simulink library "AEMS_Standard_Library"  (R2016b)
settings: Solver=ode45  StartTime=0.0  StopTime=10.0  RelTol=1e-3
undefined symbols (not defined in the file or in its folder): BkPY, carto, Cbx_extegr, Cbx_lpegrsys, Cbx_portegr, Cnx_bnk_nr_conf, Cnx_cyl_nr_conf, ConfigManagement, configuration_management, Cxx_dcm_io_tmr_end_xxxx, Cxx_dcm_rt_tmr_end, Cxx_DID_xxxx_IO_max, Cxx_DID_xxxx_IO_min, Cxx_egrhsofs, Cxx_vmaniegi, DEM_DEBOUNCE_FREEZE, DEM_DTR_CTL_INVISIBLE, DEM_DTR_CTL_NORMAL, Dem_DtrId2_XXX, Dem_DtrId3_XXX, Dem_DtrId4_XXX, Dem_DtrId5_XXX, Dem_DtrId6_XXX, Dem_DtrId7_XXX, Dem_DtrId8_XXX, Dem_DtrId9_XXX, Dem_DtrId_XXX, Dem_EnableConditionId2_XXX, Dem_EnableConditionId3_XXX, Dem_EnableConditionId4_XXX, Dem_EnableConditionId5_XXX, Dem_EnableConditionId6_XXX, Dem_EnableConditionId7_XXX, Dem_EnableConditionId8_XXX, Dem_EnableConditionId_XXX, Dem_EventId, Dem_EventId2_XXX, Dem_EventId3_XXX, Dem_EventId4_XXX, Dem_EventId5_XXX, Dem_EventId6_XXX, Dem_EventId7_XXX, Dem_EventId8_XXX, Dem_EventId9_XXX, Dem_EventId_Device_Faulttype, Dem_EventId_XXX, DEM_IUMPR_GENERAL_DENOMINATOR, DEM_OPCYC_IGNITION, Dem_RatioId2_XXX, Dem_RatioId3_XXX, Dem_RatioId4_XXX, Dem_RatioId5_XXX, Dem_RatioId6_XXX, Dem_RatioId7_XXX, Dem_RatioId8_XXX, Dem_RatioId_XXX, Dem_StorageConditionId2_XXX, Dem_StorageConditionId3_XXX, Dem_StorageConditionId4_XXX, Dem_StorageConditionId5_XXX ... (+65)
libraries: AEMS_Standard_Library x477, simulink x2
(part 12 of 39)

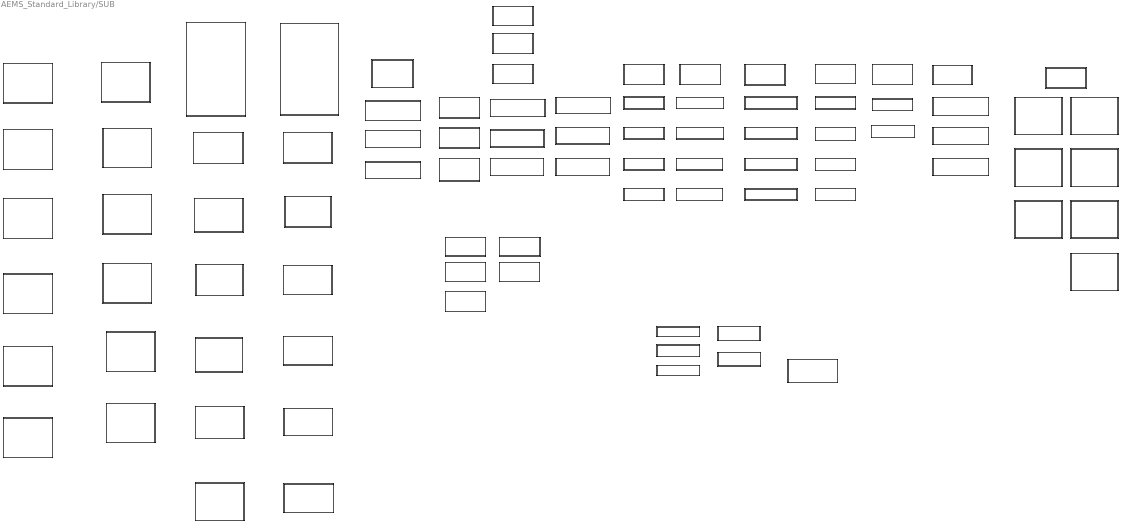
== system AEMS_Standard_Library/SUB ==
  AEMS_CONVERT_BUFFER_TO_FLP : Subsystem  Tag=[LIB]  mask(AEMS_CONVERT_BUFFER_TO_FLP){Resol=1, offset=0, DID_Datatype=int16}
      mask prompts: Resol "Resolution"; DID_Datatype "DID Datatype"
      mask help: This block converts the input buffer value to a float value.
      settings: AttributesFormatString=%<MaskType>\nResolution = %<Resol>\nOffset = %<offset>\nDIDType = %<DID_DataType>
      mask Help:
      | eval('path_lib=fileparts(which(''AEMS_Standard_Library''));');
      | doc_path = [path_lib'\help\AEMS_CONVERT_BUFFER_TO_FLP.pdf'];
      | eval('open(doc_path)');
      mask TypeOptions DID_Datatype: int8 | uint8 | int16 | uint16 | int32 | uint32
      mask Display:
      | try
      |     set_param(gcb,'MaskIconOpaque','opaque-with-ports');
      | catch
      |     set_param(gcb,'MaskIconOpaque','off');
      | end
      | 
      | disp('CONVERT_BUFFER_TO_FLP');
  AEMS_CONVERT_BYTE_TO_FLP : Subsystem  Tag=[LIB]  mask(AEMS_CONVERT_BYTE_TO_FLP){Resol=1, offset=0, DID_Datatype=int8}
      mask prompts: Resol "Resolution"; DID_Datatype "DID Datatype"
      mask help: This block is used to convert 1 byte data to corresponding floating point value based on resolution , offset & DID datatype.
      settings: AttributesFormatString=%<MaskType>\nResolution = %<Resol>\nOffset = %<offset>\nDIDType = %<DID_DataType>
      mask Help:
      | eval('path_lib=fileparts(which(''AEMS_Standard_Library''));');
      | doc_path = [path_lib'\help\AEMS_CONVERT_BYTE_TO_FLP'];
      | eval('open(doc_path)');
      mask TypeOptions DID_Datatype: int8 | uint8
      mask Display:
      | try
      |     set_param(gcb,'MaskIconOpaque','opaque-with-ports');
      | catch
      |     set_param(gcb,'MaskIconOpaque','off');
      | end
      | 
      | disp('CONVERT_BYTE_TO_FLP');
  AEMS_DEM_COUNTERBASEDDEBOUNCE : Subsystem  Tag=[LIB]  mask(AEMS_DEM_COUNTERBASEDDEBOUNCE){eventid=Dem_EventId_Device_Faulttype}
      mask prompts: eventid "Identifier of a diagnostic event (EventID)"
      mask help:
      | It  transmit the status Failed or Passed to the DEM. Accordingly, some bits of the UDS DTC status byte changes synchronously or asynchronously according to the configuration. Debounce is based on counter.
      |
      | -INPUTS-
      | conditionfulfilled: specifies whether the storage condition assigned to the StorageConditionID is fulfilled
      | prefailed: Monitor reports nonqualified test result pre-failed
      | prepassed: Monitor reports nonqualified test result pre-passed
      | reseteventdebounce: Freeze or reset the internal debounce counter/timer.
      | Dem Debounce Behavior: The event debounce counter will be frozen or reset (0 for FREEZE and 1 for RESET)
      | Dem Debounce Counter Failed Threshold: Defines the value of the internal debounce counter, which indicates the failed status.
      | Dem Debounce Counter Increment Step Size: Defines the incrementation  step size for counter (PREFAILED)
      | Dem Debounce Counter Jump Up: Activation of Jump-Up. True: activated. False: deactivated
      | Dem Debounce Counter Jump Up Value: Initialization value for the counter when PREFAILED
      | Dem Debounce Counter Passed Threshold: Defines the value of the internal debounce counter, which indicates the passed status.
      | Dem Debounce Counter Decrement Step Size: Defines the decrementation step for of counter (PREPASSED).
      | Dem Debounce Counter Jump Down: Activation of Jump-Down. True: Jump-Down activated
      | Dem Debounce Counter Jump Down Value: Initialization value for the counter when PREPASSED
      |
      | -OUTPUTS-
      | debouncevalue: Value of the debounce counter
      | failed: Diagnostic monitor reports an event Failed
      | passed: Diagnostic monitor reports an event passed
      |
      | -PARAMETERS-
      | EventID: Internal identifier of a diagnostic event. 0 is not a valid value.
      mask init:
      | eval([char(eventid) '= 0;'])
      | eventid_b = find_system(gcb,'LookUnderMasks','all','FollowLinks','on','Name','EventId_block');
      | set_param([eventid_b{:}],'Value',char(eventid));
      settings: AttributesFormatString=|
      | %<MaskType>
      | EventId: %<eventid>
  AEMS_DEM_COUNTER_BASED_DEBOUNCE_1D : Subsystem  Tag=[LIB]  Description=This subsystem is interface for self diagnosis standard calculated from similar condition and NG judgment.  mask(AEMS_DEM_COUNTER_BASED_DEBOUNCE_1D){eventid=Dem_EventId_Device_Faulttype, DemDebounceBehavior1=DEM_DEBOUNCE_FREEZE (0), DemCounterFailedThreshold=Cnx_dem_fail_thd_Device_Faulttype, DemCounterIncrementStepSize=Cnx_dem_pfail_inc_step_Device_Faulttype, DemCounterJumpUp=Cbx_dem_jmp_up_act_Device_Faulttype, DemCounterJumpUpValue=Cnx_dem_jmp_up_pfail_Device_Faulttype, DemCounterPassedThreshold=Cnx_dem_pass_thd_Device_Faulttype, DemCounterDecrementStepSize=Cnx_dem_ppass_dec_step_Device_Faulttype, DemCounterJumpDown=Cbx_dem_jmp_dwn_act_Device_Faulttype, DemCounterJumpDownValue=Cnx_dem_jmp_dwn_ppass_Device_Faulttype, DemCounterBypassFailure=Cbx_dem_byp_fail_Device_Faulttype}
      mask prompts: eventid "Identifier of a diagnostic event (EventId)"; DemDebounceBehavior1 "Dem Debounce Behavior"; DemCounterFailedThreshold "Dem Debounce Counter Failed Threshold"; DemCounterIncrementStepSize "Dem Debounce Counter Increment Step Size"; DemCounterJumpUp "Dem Debounce Counter Jump Up"; DemCounterJumpUpValue "Dem Debounce Counter Jump Up Value"; DemCounterPassedThreshold "Dem Debounce Counter Passed Threshold"; DemCounterDecrementStepSize "Dem Debounce Counter Decrement Step Size"; DemCounterJumpDown "Dem Debounce Counter Jump Down"; DemCounterJumpDownValue "Dem Debounce Counter Jump Down Value"; DemCounterBypassFailure "Dem Debounce Counter Bypass Failure"
      mask help:
      | It  transmit the status Failed or Passed to the DEM. Accordingly, some bits of the UDS DTC status byte changes synchronously or asynchronously according to the configuration. Debounce is based on counter.
      |
      | -INPUTS-
      | conditionfulfilled: specifies whether the storage condition assigned to the StorageConditionID is fulfilled
      | prefailed: Monitor reports nonqualified test result pre-failed
      | prepassed: Monitor reports nonqualified test result pre-passed
      | reseteventdebounce: Freeze or reset the internal debounce counter/timer.
      |
      | -OUTPUTS-
      | debouncevalue: Value of the debounce counter
      | failed: Diagnostic monitor reports an event Failed
      | passed: Diagnostic monitor reports an event passed
      |
      | -PARAMETERS-
      | Device: Device type
      | FaultType: Fault Type
      | EventID: Internal identifier of a diagnostic event. 0 is not a valid value.
      | Dem Debounce Behavior: The event debounce counter will be frozen or reset (0 for FREEZE and 1 for RESET)
      | Dem Debounce Counter Failed Threshold: Defines the value of the internal debounce counter, which indicates the failed status.
      | Dem Debounce Counter Increment Step Size: Defines the incrementation  step size for counter (PREFAILED)
      | Dem Debounce Counter Jump Up: Activation of Jump-Up. True: activated. False: deactivated
      | Dem Debounce Counter Jump Up Value: Initialization value for the counter when PREFAILED
      | Dem Debounce Counter Passed Threshold: Defines the value of the internal debounce counter, which indicates the passed status.
      | Dem Debounce Counter Decrement Step Size: Defines the decrementation step for of counter (PREPASSED).
      | Dem Debounce Counter Jump Down: Activation of Jump-Down. True: Jump-Down activated
      | Dem Debounce Counter Jump Down Value: Initialization value for the counter when PREPASSED
      mask init:
      | ThisBlk =gcb;
      | behaviorblk = [ThisBlk,'/DemDebounceBehavior'];
      | Bpath = [ThisBlk,'/AEMS_DEM_COUNTER_BASED_DEBOUNCE_CALL/AEMS_DEM_COUNTERBASEDDEBOUNCE'];
      | set_param(Bpath,'eventid',eventid);
      | if strcmpi(DemDebounceBehavior1,'DEM_DEBOUNCE_FREEZE (0)')
      |    set_param(behaviorblk,'Value','0');
      | elseif strcmpi(DemDebounceBehavior1,'DEM_DEBOUNCE_RESET (1)')
      |     set_param(behaviorblk,'Value','1');
      | end
      settings: AttributesFormatString=|
      | %<MaskType>
      | EventId: %<eventid>\nDem Debounce Behavior = %<DemDebounceBehavior1>\nDem Debounce Counter Failed Threshold = %<DemCounterFailedThreshold>\nDem Debounce Counter Increment Step Size = %<DemCounterIncrementStepSize>\nDem Debounce Counter Jump Up = %<DemCounterJumpUp>\nDem Debounce Counter Jump Up Value = %<DemCounterJumpUpValue>\nDem Debounce Counter Passed Threshold = %<DemCounterPassedThreshold>\nDem Debounce Counter Decrement Step Size = %<DemCounterDecrementStepSize>\nDem Debounce Counter Jump Down = %<DemCounterJumpDown>\nDem Debounce Counter Jump Down Value = %<DemCounterJumpDownValue>\nDem Debounce Counter Bypass Failure = %<DemCounterBypassFailure>
      mask Help:
      | eval('path_lib=fileparts(which(''AEMS_Standard_Library''));');
      | doc_path = [path_lib '\help\AEMS_DEM_COUNTER_BASED_DEBOUNCE.pdf'];
      | eval('open(doc_path)')
      mask TypeOptions DemDebounceBehavior1: DEM_DEBOUNCE_FREEZE (0) | DEM_DEBOUNCE_RESET (1)
  AEMS_DEM_COUNTER_BASED_DEBOUNCE_2D : Subsystem  Tag=[LIB]  Description=This subsystem is interface for self diagnosis standard calculated from similar condition and NG judgment.  mask(AEMS_DEM_COUNTER_BASED_DEBOUNCE_2D){eventid=Dem_EventId_Device_Faulttype, DemDebounceBehavior1=DEM_DEBOUNCE_FREEZE (0), DemDebounceBehavior2=DEM_DEBOUNCE_FREEZE (0), DemCounterFailedThreshold=Cnx_dem_fail_thd_Device_Faulttype, DemCounterIncrementStepSize=Cnx_dem_pfail_inc_step_Device_Faulttype, DemCounterJumpUp=Cbx_dem_jmp_up_act_Device_Faulttype, DemCounterJumpUpValue=Cnx_dem_jmp_up_pfail_Device_Faulttype, DemCounterPassedThreshold=Cnx_dem_pass_thd_Device_Faulttype, DemCounterDecrementStepSize=Cnx_dem_ppass_dec_step_Device_Faulttype, DemCounterJumpDown=Cbx_dem_jmp_dwn_act_Device_Faulttype, DemCounterJumpDownValue=Cnx_dem_jmp_dwn_ppass_Device_Faulttype, DemCounterBypassFailure=Cbx_dem_byp_fail_Device_Faulttype}
      mask prompts: eventid "Identifier of a diagnostic event (EventId)"; DemDebounceBehavior1 "Dem Debounce Behavior 1"; DemDebounceBehavior2 "Dem Debounce Behavior 2"; DemCounterFailedThreshold "Dem Debounce Counter Failed Threshold"; DemCounterIncrementStepSize "Dem Debounce Counter Increment Step Size"; DemCounterJumpUp "Dem Debounce Counter Jump Up"; DemCounterJumpUpValue "Dem Debounce Counter Jump Up Value"; DemCounterPassedThreshold "Dem Debounce Counter Passed Threshold"; DemCounterDecrementStepSize "Dem Debounce Counter Decrement Step Size"; DemCounterJumpDown "Dem Debounce Counter Jump Down"; DemCounterJumpDownValue "Dem Debounce Counter Jump Down Value"; DemCounterBypassFailure "Dem Debounce Counter Bypass Failure"
      mask help:
      | It  transmit the status Failed or Passed to the DEM. Accordingly, some bits of the UDS DTC status byte changes synchronously or asynchronously according to the configuration. Debounce is based on counter.
      |
      | -INPUTS-
      | conditionfulfilled: specifies whether the storage condition assigned to the StorageConditionID is fulfilled
      | prefailed: Monitor reports nonqualified test result pre-failed
      | prepassed: Monitor reports nonqualified test result pre-passed
      | reseteventdebounce: Freeze or reset the internal debounce counter/timer.
      |
      | -OUTPUTS-
      | debouncevalue: Value of the debounce counter
      | failed: Diagnostic monitor reports an event Failed
      | passed: Diagnostic monitor reports an event passed
      |
      | -PARAMETERS-
      | Device: Device type
      | FaultType: Fault Type
      | EventID: Internal identifier of a diagnostic event. 0 is not a valid value.
      | Dem Debounce Behavior: The event debounce counter will be frozen or reset (0 for FREEZE and 1 for RESET)
      | Dem Debounce Counter Failed Threshold: Defines the value of the internal debounce counter, which indicates the failed status.
      | Dem Debounce Counter Increment Step Size: Defines the incrementation  step size for counter (PREFAILED)
      | Dem Debounce Counter Jump Up: Activation of Jump-Up. True: activated. False: deactivated
      | Dem Debounce Counter Jump Up Value: Initialization value for the counter when PREFAILED
      | Dem Debounce Counter Passed Threshold: Defines the value of the internal debounce counter, which indicates the passed status.
      | Dem Debounce Counter Decrement Step Size: Defines the decrementation step for of counter (PREPASSED).
      | Dem Debounce Counter Jump Down: Activation of Jump-Down. True: Jump-Down activated
      | Dem Debounce Counter Jump Down Value: Initialization value for the counter when PREPASSED
      mask init:
      | ThisBlk =gcb;
      | DemDebounceBehaviors = {DemDebounceBehavior1,DemDebounceBehavior2};   
      | behaviorblk = [ThisBlk,'/DemDebounceBehavior'];
      | behaviorvector = '[';
      |     for cnt=1:2        
      |         cnt_str=num2str(cnt);
      |         Bpath = [ThisBlk,'/AEMS_DEM_COUNTER_BASED_DEBOUNCE_CALL',cnt_str,'/AEMS_DEM_COUNTERBASEDDEBOUNCE'];
      | %         set_param(Bpath,'eventid',[eventid,'_' cnt_str]);
      |         if (cnt==1)
      |             set_param(Bpath,'eventid',eventid);
      |         else
      |             Splitname=regexp(eventid,'_','all');
      |             New_EventId=insertBefore(eventid,Splitname(end),num2str(cnt));
      |             set_param(Bpath,'eventid',New_EventId);
      |         end
      |         if strcmpi(DemDebounceBehaviors{cnt},'DEM_DEBOUNCE_FREEZE (0)')
      |            behaviorvector= [behaviorvector,'0,'];
      |         else    
      |            behaviorvector= [behaviorvector,'1,'];        
      |         end
      |     end
      |     behaviorvector = behaviorvector(1:end-1);%Why end-1? I want to skip ',' for the last field.
      |     behaviorvector = [behaviorvector,']'];
      |     set_param(behaviorblk,'Value',behaviorvector);
      settings: AttributesFormatString=|
      | %<MaskType>
      | EventId: %<eventid>\nDem Debounce Behavior 1= %<DemDebounceBehavior1>\nDem Debounce Behavior 2= %<DemDebounceBehavior2>\nDem Debounce Counter Failed Threshold = %<DemCounterFailedThreshold>\nDem Debounce Counter Increment Step Size = %<DemCounterIncrementStepSize>\nDem Debounce Counter Jump Up = %<DemCounterJumpUp>\nDem Debounce Counter Jump Up Value = %<DemCounterJumpUpValue>\nDem Debounce Counter Passed Threshold = %<DemCounterPassedThreshold>\nDem Debounce Counter Decrement Step Size = %<DemCounterDecrementStepSize>\nDem Debounce Counter Jump Down = %<DemCounterJumpDown>\nDem Debounce Counter Jump Down Value = %<DemCounterJumpDownValue>\nDem Debounce Counter Bypass Failure = %<DemCounterBypassFailure>
      mask Help:
      | eval('path_lib=fileparts(which(''AEMS_Standard_Library''));');
      | doc_path = [path_lib '\help\AEMS_DEM_COUNTER_BASED_DEBOUNCE.pdf'];
      | eval('open(doc_path)')
      mask TypeOptions DemDebounceBehavior1: DEM_DEBOUNCE_FREEZE (0) | DEM_DEBOUNCE_RESET (1)
      mask TypeOptions DemDebounceBehavior2: DEM_DEBOUNCE_FREEZE (0) | DEM_DEBOUNCE_RESET (1)
  AEMS_DEM_COUNTER_BASED_DEBOUNCE_3D : Subsystem  Tag=[LIB]  Description=This subsystem is interface for self diagnosis standard calculated from similar condition and NG judgment.  mask(AEMS_DEM_COUNTER_BASED_DEBOUNCE_3D){eventid=Dem_EventId_Device_Faulttype, DemDebounceBehavior1=DEM_DEBOUNCE_FREEZE (0), DemDebounceBehavior2=DEM_DEBOUNCE_FREEZE (0), DemDebounceBehavior3=DEM_DEBOUNCE_FREEZE (0), DemCounterFailedThreshold=Cnx_dem_fail_thd_Device_Faulttype, DemCounterIncrementStepSize=Cnx_dem_pfail_inc_step_Device_Faulttype, DemCounterJumpUp=Cbx_dem_jmp_up_act_Device_Faulttype, DemCounterJumpUpValue=Cnx_dem_jmp_up_pfail_Device_Faulttype, DemCounterPassedThreshold=Cnx_dem_pass_thd_Device_Faulttype, DemCounterDecrementStepSize=Cnx_dem_ppass_dec_step_Device_Faulttype, DemCounterJumpDown=Cbx_dem_jmp_dwn_act_Device_Faulttype, DemCounterJumpDownValue=Cnx_dem_jmp_dwn_ppass_Device_Faulttype, DemCounterBypassFailure=Cbx_dem_byp_fail_Device_Faulttype}
      mask prompts: eventid "Identifier of a diagnostic event (EventId)"; DemDebounceBehavior1 "Dem Debounce Behavior 1"; DemDebounceBehavior2 "Dem Debounce Behavior 2"; DemDebounceBehavior3 "Dem Debounce Behavior 3"; DemCounterFailedThreshold "Dem Debounce Counter Failed Threshold"; DemCounterIncrementStepSize "Dem Debounce Counter Increment Step Size"; DemCounterJumpUp "Dem Debounce Counter Jump Up"; DemCounterJumpUpValue "Dem Debounce Counter Jump Up Value"; DemCounterPassedThreshold "Dem Debounce Counter Passed Threshold"; DemCounterDecrementStepSize "Dem Debounce Counter Decrement Step Size"; DemCounterJumpDown "Dem Debounce Counter Jump Down"; DemCounterJumpDownValue "Dem Debounce Counter Jump Down Value"; DemCounterBypassFailure "Dem Debounce Counter Bypass Failure"
      mask help:
      | It  transmit the status Failed or Passed to the DEM. Accordingly, some bits of the UDS DTC status byte changes synchronously or asynchronously according to the configuration. Debounce is based on counter.
      |
      | -INPUTS-
      | conditionfulfilled: specifies whether the storage condition assigned to the StorageConditionID is fulfilled
      | prefailed: Monitor reports nonqualified test result pre-failed
      | prepassed: Monitor reports nonqualified test result pre-passed
      | reseteventdebounce: Freeze or reset the internal debounce counter/timer.
      |
      | -OUTPUTS-
      | debouncevalue: Value of the debounce counter
      | failed: Diagnostic monitor reports an event Failed
      | passed: Diagnostic monitor reports an event passed
      |
      | -PARAMETERS-
      | Device: Device type
      | FaultType: Fault Type
      | EventID: Internal identifier of a diagnostic event. 0 is not a valid value.
      | Dem Debounce Behavior: The event debounce counter will be frozen or reset (0 for FREEZE and 1 for RESET)
      | Dem Debounce Counter Failed Threshold: Defines the value of the internal debounce counter, which indicates the failed status.
      | Dem Debounce Counter Increment Step Size: Defines the incrementation  step size for counter (PREFAILED)
      | Dem Debounce Counter Jump Up: Activation of Jump-Up. True: activated. False: deactivated
      | Dem Debounce Counter Jump Up Value: Initialization value for the counter when PREFAILED
      | Dem Debounce Counter Passed Threshold: Defines the value of the internal debounce counter, which indicates the passed status.
      | Dem Debounce Counter Decrement Step Size: Defines the decrementation step for of counter (PREPASSED).
      | Dem Debounce Counter Jump Down: Activation of Jump-Down. True: Jump-Down activated
      | Dem Debounce Counter Jump Down Value: Initialization value for the counter when PREPASSED
      mask init:
      | ThisBlk =gcb;
      | DemDebounceBehaviors = {DemDebounceBehavior1,DemDebounceBehavior2,DemDebounceBehavior3};   
      | behaviorblk = [ThisBlk,'/DemDebounceBehavior'];
      | behaviorvector = '[';
      |     for cnt=1:3        
      |         cnt_str=num2str(cnt);
      |         Bpath = [ThisBlk,'/AEMS_DEM_COUNTER_BASED_DEBOUNCE_CALL',cnt_str,'/AEMS_DEM_COUNTERBASEDDEBOUNCE'];
      |  %         set_param(Bpath,'eventid',[eventid,'_' cnt_str]);
      |         if (cnt==1)
      |             set_param(Bpath,'eventid',eventid);
      |         else
      |             Splitname=regexp(eventid,'_','all');
      |             New_EventId=insertBefore(eventid,Splitname(end),num2str(cnt));
      |             set_param(Bpath,'eventid',New_EventId);
      |         end
      |         if strcmpi(DemDebounceBehaviors{cnt},'DEM_DEBOUNCE_FREEZE (0)')
      |            behaviorvector= [behaviorvector,'0,'];
      |         else    
      |            behaviorvector= [behaviorvector,'1,'];        
      |         end
      |     end
      |     behaviorvector = behaviorvector(1:end-1);%Why end-1? I want to skip ',' for the last field.
      |     behaviorvector = [behaviorvector,']'];
      |     set_param(behaviorblk,'Value',behaviorvector);
      settings: AttributesFormatString=|
      | %<MaskType>
      | EventId: %<eventid>\nDem Debounce Behavior 1= %<DemDebounceBehavior1>\nDem Debounce Behavior 2= %<DemDebounceBehavior2>\nDem Debounce Behavior 3= %<DemDebounceBehavior3>\nDem Debounce Counter Failed Threshold = %<DemCounterFailedThreshold>\nDem Debounce Counter Increment Step Size = %<DemCounterIncrementStepSize>\nDem Debounce Counter Jump Up = %<DemCounterJumpUp>\nDem Debounce Counter Jump Up Value = %<DemCounterJumpUpValue>\nDem Debounce Counter Passed Threshold = %<DemCounterPassedThreshold>\nDem Debounce Counter Decrement Step Size = %<DemCounterDecrementStepSize>\nDem Debounce Counter Jump Down = %<DemCounterJumpDown>\nDem Debounce Counter Jump Down Value = %<DemCounterJumpDownValue>\nDem Debounce Counter Bypass Failure = %<DemCounterBypassFailure>
      mask Help:
      | eval('path_lib=fileparts(which(''AEMS_Standard_Library''));');
      | doc_path = [path_lib '\help\AEMS_DEM_COUNTER_BASED_DEBOUNCE.pdf'];
      | eval('open(doc_path)')
      mask TypeOptions DemDebounceBehavior1: DEM_DEBOUNCE_FREEZE (0) | DEM_DEBOUNCE_RESET (1)
      mask TypeOptions DemDebounceBehavior2: DEM_DEBOUNCE_FREEZE (0) | DEM_DEBOUNCE_RESET (1)
      mask TypeOptions DemDebounceBehavior3: DEM_DEBOUNCE_FREEZE (0) | DEM_DEBOUNCE_RESET (1)
  AEMS_DEM_COUNTER_BASED_DEBOUNCE_4D : Subsystem  Tag=[LIB]  Description=This subsystem is interface for self diagnosis standard calculated from similar condition and NG judgment.  mask(AEMS_DEM_COUNTER_BASED_DEBOUNCE_4D){eventid=Dem_EventId_Device_Faulttype, DemDebounceBehavior1=DEM_DEBOUNCE_FREEZE (0), DemDebounceBehavior2=DEM_DEBOUNCE_FREEZE (0), DemDebounceBehavior3=DEM_DEBOUNCE_FREEZE (0), DemDebounceBehavior4=DEM_DEBOUNCE_FREEZE (0), DemCounterFailedThreshold=Cnx_dem_fail_thd_Device_Faulttype, DemCounterIncrementStepSize=Cnx_dem_pfail_inc_step_Device_Faulttype, DemCounterJumpUp=Cbx_dem_jmp_up_act_Device_Faulttype, DemCounterJumpUpValue=Cnx_dem_jmp_up_pfail_Device_Faulttype, DemCounterPassedThreshold=Cnx_dem_pass_thd_Device_Faulttype, DemCounterDecrementStepSize=Cnx_dem_ppass_dec_step_Device_Faulttype, DemCounterJumpDown=Cbx_dem_jmp_dwn_act_Device_Faulttype, DemCounterJumpDownValue=Cnx_dem_jmp_dwn_ppass_Device_Faulttype, DemCounterBypassFailure=Cbx_dem_byp_fail_Device_Faulttype}
      mask prompts: eventid "Identifier of a diagnostic event (EventId)"; DemDebounceBehavior1 "Dem Debounce Behavior 1"; DemDebounceBehavior2 "Dem Debounce Behavior 2"; DemDebounceBehavior3 "Dem Debounce Behavior 3"; DemDebounceBehavior4 "Dem Debounce Behavior 4"; DemCounterFailedThreshold "Dem Debounce Counter Failed Threshold"; DemCounterIncrementStepSize "Dem Debounce Counter Increment Step Size"; DemCounterJumpUp "Dem Debounce Counter Jump Up"; DemCounterJumpUpValue "Dem Debounce Counter Jump Up Value"; DemCounterPassedThreshold "Dem Debounce Counter Passed Threshold"; DemCounterDecrementStepSize "Dem Debounce Counter Decrement Step Size"; DemCounterJumpDown "Dem Debounce Counter Jump Down"; DemCounterJumpDownValue "Dem Debounce Counter Jump Down Value"; DemCounterBypassFailure "Dem Debounce Counter Bypass Failure"
      mask help:
      | It  transmit the status Failed or Passed to the DEM. Accordingly, some bits of the UDS DTC status byte changes synchronously or asynchronously according to the configuration. Debounce is based on counter.
      |
      | -INPUTS-
      | conditionfulfilled: specifies whether the storage condition assigned to the StorageConditionID is fulfilled
      | prefailed: Monitor reports nonqualified test result pre-failed
      | prepassed: Monitor reports nonqualified test result pre-passed
      | reseteventdebounce: Freeze or reset the internal debounce counter/timer.
      |
      | -OUTPUTS-
      | debouncevalue: Value of the debounce counter
      | failed: Diagnostic monitor reports an event Failed
      | passed: Diagnostic monitor reports an event passed
      |
      | -PARAMETERS-
      | Device: Device type
      | FaultType: Fault Type
      | EventID: Internal identifier of a diagnostic event. 0 is not a valid value.
      | Dem Debounce Behavior: The event debounce counter will be frozen or reset (0 for FREEZE and 1 for RESET)
      | Dem Debounce Counter Failed Threshold: Defines the value of the internal debounce counter, which indicates the failed status.
      | Dem Debounce Counter Increment Step Size: Defines the incrementation  step size for counter (PREFAILED)
      | Dem Debounce Counter Jump Up: Activation of Jump-Up. True: activated. False: deactivated
      | Dem Debounce Counter Jump Up Value: Initialization value for the counter when PREFAILED
      | Dem Debounce Counter Passed Threshold: Defines the value of the internal debounce counter, which indicates the passed status.
      | Dem Debounce Counter Decrement Step Size: Defines the decrementation step for of counter (PREPASSED).
      | Dem Debounce Counter Jump Down: Activation of Jump-Down. True: Jump-Down activated
      | Dem Debounce Counter Jump Down Value: Initialization value for the counter when PREPASSED
      mask init:
      | ThisBlk =gcb;
      | DemDebounceBehaviors = {DemDebounceBehavior1,DemDebounceBehavior2,DemDebounceBehavior3,DemDebounceBehavior4};   
      | behaviorblk = [ThisBlk,'/DemDebounceBehavior'];
      | behaviorvector = '[';
      |     for cnt=1:4        
      |         cnt_str=num2str(cnt);
      |         Bpath = [ThisBlk,'/AEMS_DEM_COUNTER_BASED_DEBOUNCE_CALL',cnt_str,'/AEMS_DEM_COUNTERBASEDDEBOUNCE'];
      | %         set_param(Bpath,'eventid',[eventid,'_' cnt_str]);
      |         if (cnt==1)
      |             set_param(Bpath,'eventid',eventid);
      |         else
      |             Splitname=regexp(eventid,'_','all');
      |             New_EventId=insertBefore(eventid,Splitname(end),num2str(cnt));
      |             set_param(Bpath,'eventid',New_EventId);
      |         end
      |         if strcmpi(DemDebounceBehaviors{cnt},'DEM_DEBOUNCE_FREEZE (0)')
      |            behaviorvector= [behaviorvector,'0,'];
      |         else    
      |            behaviorvector= [behaviorvector,'1,'];        
      |         end
      |     end
      |     behaviorvector = behaviorvector(1:end-1);%Why end-1? I want to skip ',' for the last field.
      |     behaviorvector = [behaviorvector,']'];
      |     set_param(behaviorblk,'Value',behaviorvector);
      settings: AttributesFormatString=|
      | %<MaskType>
      | EventId: %<eventid>\nDem Debounce Behavior 1= %<DemDebounceBehavior1>\nDem Debounce Behavior 2= %<DemDebounceBehavior2>\nDem Debounce Behavior 3= %<DemDebounceBehavior3>\nDem Debounce Behavior 4= %<DemDebounceBehavior4>\nDem Debounce Counter Failed Threshold = %<DemCounterFailedThreshold>\nDem Debounce Counter Increment Step Size = %<DemCounterIncrementStepSize>\nDem Debounce Counter Jump Up = %<DemCounterJumpUp>\nDem Debounce Counter Jump Up Value = %<DemCounterJumpUpValue>\nDem Debounce Counter Passed Threshold = %<DemCounterPassedThreshold>\nDem Debounce Counter Decrement Step Size = %<DemCounterDecrementStepSize>\nDem Debounce Counter Jump Down = %<DemCounterJumpDown>\nDem Debounce Counter Jump Down Value = %<DemCounterJumpDownValue>\nDem Debounce Counter Bypass Failure = %<DemCounterBypassFailure>
      mask Help:
      | eval('path_lib=fileparts(which(''AEMS_Standard_Library''));');
      | doc_path = [path_lib '\help\AEMS_DEM_COUNTER_BASED_DEBOUNCE.pdf'];
      | eval('open(doc_path)')
      mask TypeOptions DemDebounceBehavior1: DEM_DEBOUNCE_FREEZE (0) | DEM_DEBOUNCE_RESET (1)
      mask TypeOptions DemDebounceBehavior2: DEM_DEBOUNCE_FREEZE (0) | DEM_DEBOUNCE_RESET (1)
      mask TypeOptions DemDebounceBehavior3: DEM_DEBOUNCE_FREEZE (0) | DEM_DEBOUNCE_RESET (1)
      mask TypeOptions DemDebounceBehavior4: DEM_DEBOUNCE_FREEZE (0) | DEM_DEBOUNCE_RESET (1)
  AEMS_DEM_COUNTER_BASED_DEBOUNCE_6D : Subsystem  Tag=[LIB]  Description=This subsystem is interface for self diagnosis standard calculated from similar condition and NG judgment.  mask(AEMS_DEM_COUNTER_BASED_DEBOUNCE_6D){eventid=Dem_EventId_Device_Faulttype, DemDebounceBehavior1=DEM_DEBOUNCE_FREEZE (0), DemDebounceBehavior2=DEM_DEBOUNCE_FREEZE (0), DemDebounceBehavior3=DEM_DEBOUNCE_FREEZE (0), DemDebounceBehavior4=DEM_DEBOUNCE_FREEZE (0), DemDebounceBehavior5=DEM_DEBOUNCE_FREEZE (0), DemDebounceBehavior6=DEM_DEBOUNCE_FREEZE (0), DemCounterFailedThreshold=Cnx_dem_fail_thd_Device_Faulttype, DemCounterIncrementStepSize=Cnx_dem_pfail_inc_step_Device_Faulttype, DemCounterJumpUp=Cbx_dem_jmp_up_act_Device_Faulttype, DemCounterJumpUpValue=Cnx_dem_jmp_up_pfail_Device_Faulttype, DemCounterPassedThreshold=Cnx_dem_pass_thd_Device_Faulttype, DemCounterDecrementStepSize=Cnx_dem_ppass_dec_step_Device_Faulttype, DemCounterJumpDown=Cbx_dem_jmp_dwn_act_Device_Faulttype, DemCounterJumpDownValue=Cnx_dem_jmp_dwn_ppass_Device_Faulttype, DemCounterBypassFailure=Cbx_dem_byp_fail_Device_Faulttype}
      mask prompts: eventid "Identifier of a diagnostic event (EventId)"; DemDebounceBehavior1 "Dem Debounce Behavior 1"; DemDebounceBehavior2 "Dem Debounce Behavior 2"; DemDebounceBehavior3 "Dem Debounce Behavior 3"; DemDebounceBehavior4 "Dem Debounce Behavior 4"; DemDebounceBehavior5 "Dem Debounce Behavior 5"; DemDebounceBehavior6 "Dem Debounce Behavior 6"; DemCounterFailedThreshold "Dem Debounce Counter Failed Threshold"; DemCounterIncrementStepSize "Dem Debounce Counter Increment Step Size"; DemCounterJumpUp "Dem Debounce Counter Jump Up"; DemCounterJumpUpValue "Dem Debounce Counter Jump Up Value"; DemCounterPassedThreshold "Dem Debounce Counter Passed Threshold"; DemCounterDecrementStepSize "Dem Debounce Counter Decrement Step Size"; DemCounterJumpDown "Dem Debounce Counter Jump Down"; DemCounterJumpDownValue "Dem Debounce Counter Jump Down Value"; DemCounterBypassFailure "Dem Debounce Counter Bypass Failure"
      mask help:
      | It  transmit the status Failed or Passed to the DEM. Accordingly, some bits of the UDS DTC status byte changes synchronously or asynchronously according to the configuration. Debounce is based on counter.
      |
      | -INPUTS-
      | conditionfulfilled: specifies whether the storage condition assigned to the StorageConditionID is fulfilled
      | prefailed: Monitor reports nonqualified test result pre-failed
      | prepassed: Monitor reports nonqualified test result pre-passed
      | reseteventdebounce: Freeze or reset the internal debounce counter/timer.
      |
      | -OUTPUTS-
      | debouncevalue: Value of the debounce counter
      | failed: Diagnostic monitor reports an event Failed
      | passed: Diagnostic monitor reports an event passed
      |
      | -PARAMETERS-
      | Device: Device type
      | FaultType: Fault Type
      | EventID: Internal identifier of a diagnostic event. 0 is not a valid value.
      | Dem Debounce Behavior: The event debounce counter will be frozen or reset (0 for FREEZE and 1 for RESET)
      | Dem Debounce Counter Failed Threshold: Defines the value of the internal debounce counter, which indicates the failed status.
      | Dem Debounce Counter Increment Step Size: Defines the incrementation  step size for counter (PREFAILED)
      | Dem Debounce Counter Jump Up: Activation of Jump-Up. True: activated. False: deactivated
      | Dem Debounce Counter Jump Up Value: Initialization value for the counter when PREFAILED
      | Dem Debounce Counter Passed Threshold: Defines the value of the internal debounce counter, which indicates the passed status.
      | Dem Debounce Counter Decrement Step Size: Defines the decrementation step for of counter (PREPASSED).
      | Dem Debounce Counter Jump Down: Activation of Jump-Down. True: Jump-Down activated
      | Dem Debounce Counter Jump Down Value: Initialization value for the counter when PREPASSED
      mask init:
      | ThisBlk =gcb;
      | DemDebounceBehaviors = {DemDebounceBehavior1,DemDebounceBehavior2,DemDebounceBehavior3,DemDebounceBehavior4,DemDebounceBehavior5,DemDebounceBehavior6};   
      | behaviorblk = [ThisBlk,'/DemDebounceBehavior'];
      | behaviorvector = '[';
      |     for cnt=1:6        
      |         cnt_str=num2str(cnt);
      |         Bpath = [ThisBlk,'/AEMS_DEM_COUNTER_BASED_DEBOUNCE_CALL',cnt_str,'/AEMS_DEM_COUNTERBASEDDEBOUNCE'];
      | %         set_param(Bpath,'eventid',[eventid,'_' cnt_str]);
      |         if (cnt==1)
      |             set_param(Bpath,'eventid',eventid);
      |         else
      |             Splitname=regexp(eventid,'_','all');
      |             New_EventId=insertBefore(eventid,Splitname(end),num2str(cnt));
      |             set_param(Bpath,'eventid',New_EventId);
      |         end
      |         if strcmpi(DemDebounceBehaviors{cnt},'DEM_DEBOUNCE_FREEZE (0)')
      |            behaviorvector= [behaviorvector,'0,'];
      |         else    
      |            behaviorvector= [behaviorvector,'1,'];        
      |         end
      |     end
      |     behaviorvector = behaviorvector(1:end-1);%Why end-1? I want to skip ',' for the last field.
      |     behaviorvector = [behaviorvector,']'];
      |     set_param(behaviorblk,'Value',behaviorvector);
      settings: AttributesFormatString=|
      | %<MaskType>
      | EventId: %<eventid>\nDem Debounce Behavior 1= %<DemDebounceBehavior1>\nDem Debounce Behavior 2= %<DemDebounceBehavior2>\nDem Debounce Behavior 3= %<DemDebounceBehavior3>\nDem Debounce Behavior 4= %<DemDebounceBehavior4>\nDem Debounce Behavior 5= %<DemDebounceBehavior5>\nDem Debounce Behavior 6= %<DemDebounceBehavior6>\nDem Debounce Counter Failed Threshold = %<DemCounterFailedThreshold>\nDem Debounce Counter Increment Step Size = %<DemCounterIncrementStepSize>\nDem Debounce Counter Jump Up = %<DemCounterJumpUp>\nDem Debounce Counter Jump Up Value = %<DemCounterJumpUpValue>\nDem Debounce Counter Passed Threshold = %<DemCounterPassedThreshold>\nDem Debounce Counter Decrement Step Size = %<DemCounterDecrementStepSize>\nDem Debounce Counter Jump Down = %<DemCounterJumpDown>\nDem Debounce Counter Jump Down Value = %<DemCounterJumpDownValue>\nDem Debounce Counter Bypass Failure = %<DemCounterBypassFailure>
      mask Help:
      | eval('path_lib=fileparts(which(''AEMS_Standard_Library''));');
      | doc_path = [path_lib '\help\AEMS_DEM_COUNTER_BASED_DEBOUNCE.pdf'];
      | eval('open(doc_path)')
      mask TypeOptions DemDebounceBehavior1: DEM_DEBOUNCE_FREEZE (0) | DEM_DEBOUNCE_RESET (1)
      mask TypeOptions DemDebounceBehavior2: DEM_DEBOUNCE_FREEZE (0) | DEM_DEBOUNCE_RESET (1)
      mask TypeOptions DemDebounceBehavior3: DEM_DEBOUNCE_FREEZE (0) | DEM_DEBOUNCE_RESET (1)
      mask TypeOptions DemDebounceBehavior4: DEM_DEBOUNCE_FREEZE (0) | DEM_DEBOUNCE_RESET (1)
      mask TypeOptions DemDebounceBehavior5: DEM_DEBOUNCE_FREEZE (0) | DEM_DEBOUNCE_RESET (1)
      mask TypeOptions DemDebounceBehavior6: DEM_DEBOUNCE_FREEZE (0) | DEM_DEBOUNCE_RESET (1)
  AEMS_DEM_COUNTER_BASED_DEBOUNCE_8D : Subsystem  Tag=[LIB]  Description=This subsystem is interface for self diagnosis standard calculated from similar condition and NG judgment.  mask(AEMS_DEM_COUNTER_BASED_DEBOUNCE_8D){eventid=Dem_EventId_Device_Faulttype, DemDebounceBehavior1=DEM_DEBOUNCE_FREEZE (0), DemDebounceBehavior2=DEM_DEBOUNCE_FREEZE (0), DemDebounceBehavior3=DEM_DEBOUNCE_FREEZE (0), DemDebounceBehavior4=DEM_DEBOUNCE_FREEZE (0), DemDebounceBehavior5=DEM_DEBOUNCE_FREEZE (0), DemDebounceBehavior6=DEM_DEBOUNCE_FREEZE (0), DemDebounceBehavior7=DEM_DEBOUNCE_FREEZE (0), DemDebounceBehavior8=DEM_DEBOUNCE_FREEZE (0), DemCounterFailedThreshold=Cnx_dem_fail_thd_Device_Faulttype, DemCounterIncrementStepSize=Cnx_dem_pfail_inc_step_Device_Faulttype, DemCounterJumpUp=Cbx_dem_jmp_up_act_Device_Faulttype, DemCounterJumpUpValue=Cnx_dem_jmp_up_pfail_Device_Faulttype, DemCounterPassedThreshold=Cnx_dem_pass_thd_Device_Faulttype, DemCounterDecrementStepSize=Cnx_dem_ppass_dec_step_Device_Faulttype, DemCounterJumpDown=Cbx_dem_jmp_dwn_act_Device_Faulttype, DemCounterJumpDownValue=Cnx_dem_jmp_dwn_ppass_Device_Faulttype, DemCounterBypassFailure=Cbx_dem_byp_fail_Device_Faulttype}
      mask prompts: eventid "Identifier of a diagnostic event (EventId)"; DemDebounceBehavior1 "Dem Debounce Behavior 1"; DemDebounceBehavior2 "Dem Debounce Behavior 2"; DemDebounceBehavior3 "Dem Debounce Behavior 3"; DemDebounceBehavior4 "Dem Debounce Behavior 4"; DemDebounceBehavior5 "Dem Debounce Behavior 5"; DemDebounceBehavior6 "Dem Debounce Behavior 6"; DemDebounceBehavior7 "Dem Debounce Behavior 7"; DemDebounceBehavior8 "Dem Debounce Behavior 8"; DemCounterFailedThreshold "Dem Debounce Counter Failed Threshold"; DemCounterIncrementStepSize "Dem Debounce Counter Increment Step Size"; DemCounterJumpUp "Dem Debounce Counter Jump Up"; DemCounterJumpUpValue "Dem Debounce Counter Jump Up Value"; DemCounterPassedThreshold "Dem Debounce Counter Passed Threshold"; DemCounterDecrementStepSize "Dem Debounce Counter Decrement Step Size"; DemCounterJumpDown "Dem Debounce Counter Jump Down"; DemCounterJumpDownValue "Dem Debounce Counter Jump Down Value"; DemCounterBypassFailure "Dem Debounce Counter Bypass Failure"
      mask help:
      | It  transmit the status Failed or Passed to the DEM. Accordingly, some bits of the UDS DTC status byte changes synchronously or asynchronously according to the configuration. Debounce is based on counter.
      |
      | -INPUTS-
      | conditionfulfilled: specifies whether the storage condition assigned to the StorageConditionID is fulfilled
      | prefailed: Monitor reports nonqualified test result pre-failed
      | prepassed: Monitor reports nonqualified test result pre-passed
      | reseteventdebounce: Freeze or reset the internal debounce counter/timer.
      |
      | -OUTPUTS-
      | debouncevalue: Value of the debounce counter
      | failed: Diagnostic monitor reports an event Failed
      | passed: Diagnostic monitor reports an event passed
      |
      | -PARAMETERS-
      | Device: Device type
      | FaultType: Fault Type
      | EventID: Internal identifier of a diagnostic event. 0 is not a valid value.
      | Dem Debounce Behavior: The event debounce counter will be frozen or reset (0 for FREEZE and 1 for RESET)
      | Dem Debounce Counter Failed Threshold: Defines the value of the internal debounce counter, which indicates the failed status.
      | Dem Debounce Counter Increment Step Size: Defines the incrementation  step size for counter (PREFAILED)
      | Dem Debounce Counter Jump Up: Activation of Jump-Up. True: activated. False: deactivated
      | Dem Debounce Counter Jump Up Value: Initialization value for the counter when PREFAILED
      | Dem Debounce Counter Passed Threshold: Defines the value of the internal debounce counter, which indicates the passed status.
      | Dem Debounce Counter Decrement Step Size: Defines the decrementation step for of counter (PREPASSED).
      | Dem Debounce Counter Jump Down: Activation of Jump-Down. True: Jump-Down activated
      | Dem Debounce Counter Jump Down Value: Initialization value for the counter when PREPASSED
      mask init:
      | ThisBlk =gcb;
      | DemDebounceBehaviors = {DemDebounceBehavior1,DemDebounceBehavior2,DemDebounceBehavior3,DemDebounceBehavior4,DemDebounceBehavior5,DemDebounceBehavior6,DemDebounceBehavior7,DemDebounceBehavior8};   
      | behaviorblk = [ThisBlk,'/DemDebounceBehavior'];
      | behaviorvector = '[';
      |     for cnt=1:8        
      |         cnt_str=num2str(cnt);
      |         Bpath = [ThisBlk,'/AEMS_DEM_COUNTER_BASED_DEBOUNCE_CALL',cnt_str,'/AEMS_DEM_COUNTERBASEDDEBOUNCE'];
      | %         set_param(Bpath,'eventid',[eventid,'_' cnt_str]);
      |         if (cnt==1)
      |             set_param(Bpath,'eventid',eventid);
      |         else
      |             Splitname=regexp(eventid,'_','all');
      |             New_EventId=insertBefore(eventid,Splitname(end),num2str(cnt));
      |             set_param(Bpath,'eventid',New_EventId);
      |         end
      |         if strcmpi(DemDebounceBehaviors{cnt},'DEM_DEBOUNCE_FREEZE (0)')
      |            behaviorvector= [behaviorvector,'0,'];
      |         else    
      |            behaviorvector= [behaviorvector,'1,'];        
      |         end
      |     end
      |     behaviorvector = behaviorvector(1:end-1);%Why end-1? I want to skip ',' for the last field.
      |     behaviorvector = [behaviorvector,']'];
      |     set_param(behaviorblk,'Value',behaviorvector);
      settings: AttributesFormatString=|
      | %<MaskType>
      | EventId: %<eventid>\nDem Debounce Behavior 1= %<DemDebounceBehavior1>\nDem Debounce Behavior 2= %<DemDebounceBehavior2>\nDem Debounce Behavior 3= %<DemDebounceBehavior3>\nDem Debounce Behavior 4= %<DemDebounceBehavior4>\nDem Debounce Behavior 5= %<DemDebounceBehavior5>\nDem Debounce Behavior 6= %<DemDebounceBehavior6>\nDem Debounce Behavior 7= %<DemDebounceBehavior7>\nDem Debounce Behavior 8= %<DemDebounceBehavior8>\nDem Debounce Counter Failed Threshold = %<DemCounterFailedThreshold>\nDem Debounce Counter Increment Step Size = %<DemCounterIncrementStepSize>\nDem Debounce Counter Jump Up = %<DemCounterJumpUp>\nDem Debounce Counter Jump Up Value = %<DemCounterJumpUpValue>\nDem Debounce Counter Passed Threshold = %<DemCounterPassedThreshold>\nDem Debounce Counter Decrement Step Size = %<DemCounterDecrementStepSize>\nDem Debounce Counter Jump Down = %<DemCounterJumpDown>\nDem Debounce Counter Jump Down Value = %<DemCounterJumpDownValue>\nDem Debounce Counter Bypass Failure = %<DemCounterBypassFailure>
      mask Help:
      | eval('path_lib=fileparts(which(''AEMS_Standard_Library''));');
      | doc_path = [path_lib '\help\AEMS_DEM_COUNTER_BASED_DEBOUNCE.pdf'];
      | eval('open(doc_path)')
      mask TypeOptions DemDebounceBehavior1: DEM_DEBOUNCE_FREEZE (0) | DEM_DEBOUNCE_RESET (1)
      mask TypeOptions DemDebounceBehavior2: DEM_DEBOUNCE_FREEZE (0) | DEM_DEBOUNCE_RESET (1)
      mask TypeOptions DemDebounceBehavior3: DEM_DEBOUNCE_FREEZE (0) | DEM_DEBOUNCE_RESET (1)
      mask TypeOptions DemDebounceBehavior4: DEM_DEBOUNCE_FREEZE (0) | DEM_DEBOUNCE_RESET (1)
      mask TypeOptions DemDebounceBehavior5: DEM_DEBOUNCE_FREEZE (0) | DEM_DEBOUNCE_RESET (1)
      mask TypeOptions DemDebounceBehavior6: DEM_DEBOUNCE_FREEZE (0) | DEM_DEBOUNCE_RESET (1)
      mask TypeOptions DemDebounceBehavior7: DEM_DEBOUNCE_FREEZE (0) | DEM_DEBOUNCE_RESET (1)
      mask TypeOptions DemDebounceBehavior8: DEM_DEBOUNCE_FREEZE (0) | DEM_DEBOUNCE_RESET (1)
  AEMS_DEM_COUNTER_BASED_DEBOUNCE_THRSHOLD_DYN_1D : Subsystem  Tag=[LIB]  Description=This subsystem is interface for self diagnosis standard calculated from similar condition and NG judgment.  mask(AEMS_DEM_COUNTER_BASED_DEBOUNCE_THRSHOLD_DYN_1D){eventid=Dem_EventId_Device_Faulttype, DemDebounceBehavior1=DEM_DEBOUNCE_FREEZE (0), DemCounterIncrementStepSize=Cnx_dem_pfail_inc_step_Device_Faulttype, DemCounterJumpUp=Cbx_dem_jmp_up_act_Device_Faulttype, DemCounterJumpUpValue=Cnx_dem_jmp_up_pfail_Device_Faulttype, DemCounterDecrementStepSize=Cnx_dem_ppass_dec_step_Device_Faulttype, DemCounterJumpDown=Cbx_dem_jmp_dwn_act_Device_Faulttype, DemCounterJumpDownValue=Cnx_dem_jmp_dwn_ppass_Device_Faulttype, DemCounterBypassFailure=Cbx_dem_byp_fail_Device_Faulttype}
      mask prompts: eventid "Identifier of a diagnostic event (EventId)"; DemDebounceBehavior1 "Dem Debounce Behavior"; DemCounterIncrementStepSize "Dem Debounce Counter Increment Step Size"; DemCounterJumpUp "Dem Debounce Counter Jump Up"; DemCounterJumpUpValue "Dem Debounce Counter Jump Up Value"; DemCounterDecrementStepSize "Dem Debounce Counter Decrement Step Size"; DemCounterJumpDown "Dem Debounce Counter Jump Down"; DemCounterJumpDownValue "Dem Debounce Counter Jump Down Value"; DemCounterBypassFailure "Dem Debounce Counter Bypass Failure"
      mask help:
      | It  transmit the status Failed or Passed to the DEM. Accordingly, some bits of the UDS DTC status byte changes synchronously or asynchronously according to the configuration. Debounce is based on counter.
      |
      | -INPUTS-
      | conditionfulfilled: specifies whether the storage condition assigned to the StorageConditionID is fulfilled
      | prefailed: Monitor reports nonqualified test result pre-failed
      | prepassed: Monitor reports nonqualified test result pre-passed
      | failedthreshold: Defines the value of the internal debounce counter, which indicates the failed status.
      | passedthreshold: Defines the value of the internal debounce counter, which indicates the passed status.
      | reseteventdebounce: Freeze or reset the internal debounce counter/timer.
      |
      | -OUTPUTS-
      | debouncevalue: Value of the debounce counter
      | failed: Diagnostic monitor reports an event Failed
      | passed: Diagnostic monitor reports an event passed
      |
      | -PARAMETERS-
      | EventID: Internal identifier of a diagnostic event. 0 is not a valid value.
      | Dem Debounce Behavior: The event debounce counter will be frozen or reset (0 for FREEZE and 1 for RESET)
      | Dem Debounce Counter Increment Step Size: Defines the incrementation  step size for counter (PREFAILED)
      | Dem Debounce Counter Jump Up: Activation of Jump-Up. True: activated. False: deactivated
      | Dem Debounce Counter Jump Up Value: Initialization value for the counter when PREFAILED
      | Dem Debounce Counter Decrement Step Size: Defines the decrementation step for of counter (PREPASSED).
      | Dem Debounce Counter Jump Down: Activation of Jump-Down. True: Jump-Down activated
      | Dem Debounce Counter Jump Down Value: Initialization value for the counter when PREPASSED
      mask init:
      | ThisBlk =gcb;
      | behaviorblk = [ThisBlk,'/DemDebounceBehavior'];
      | Bpath = [ThisBlk,'/AEMS_DEM_COUNTER_BASED_DEBOUNCE_THRSHOLD_DYN_CALL/AEMS_DEM_COUNTERBASEDDEBOUNCE'];
      | set_param(Bpath,'eventid',eventid);
      | if strcmpi(DemDebounceBehavior1,'DEM_DEBOUNCE_FREEZE (0)')
      |    set_param(behaviorblk,'Value','0');
      | elseif strcmpi(DemDebounceBehavior1,'DEM_DEBOUNCE_RESET (1)')
      |     set_param(behaviorblk,'Value','1');
      | end
      settings: AttributesFormatString=|
      | %<MaskType>\nEventId: %<eventid>
      | Dem Debounce Behavior = %<DemDebounceBehavior1>
      | Dem Debounce Counter Increment Step Size = %<DemCounterIncrementStepSize>
      | Dem Debounce Counter Jump Up = %<DemCounterJumpUp>
      | Dem Debounce Counter Jump Up Value = %<DemCounterJumpUpValue>
      | Dem Debounce Counter Decrement Step Size = %<DemCounterDecrementStepSize>
      | Dem Debounce Counter Jump Down = %<DemCounterJumpDown>
      | Dem Debounce Counter Jump Down Value = %<DemCounterJumpDownValue>
      | Dem Debounce Counter Bypass Failure = %<DemCounterBypassFailure>
      mask Help:
      | eval('path_lib=fileparts(which(''AEMS_Standard_Library''));');
      | doc_path = [path_lib '\help\AEMS_DEM_COUNTER_BASED_DEBOUNCE_THRSHOLD_DYN.pdf'];
      | eval('open(doc_path)')
      mask TypeOptions DemDebounceBehavior1: DEM_DEBOUNCE_FREEZE (0) | DEM_DEBOUNCE_RESET (1)
  AEMS_DEM_COUNTER_BASED_DEBOUNCE_THRSHOLD_DYN_2D : Subsystem  Tag=[LIB]  Description=This subsystem is interface for self diagnosis standard calculated from similar condition and NG judgment.  mask(AEMS_DEM_COUNTER_BASED_DEBOUNCE_THRSHOLD_DYN_2D){eventid=Dem_EventId_Device_Faulttype, DemDebounceBehavior1=DEM_DEBOUNCE_FREEZE (0), DemDebounceBehavior2=DEM_DEBOUNCE_FREEZE (0), DemCounterIncrementStepSize=Cnx_dem_pfail_inc_step_Device_Faulttype, DemCounterJumpUp=Cbx_dem_jmp_up_act_Device_Faulttype, DemCounterJumpUpValue=Cnx_dem_jmp_up_pfail_Device_Faulttype, DemCounterDecrementStepSize=Cnx_dem_ppass_dec_step_Device_Faulttype, DemCounterJumpDown=Cbx_dem_jmp_dwn_act_Device_Faulttype, DemCounterJumpDownValue=Cnx_dem_jmp_dwn_ppass_Device_Faulttype, DemCounterBypassFailure=Cbx_dem_byp_fail_Device_Faulttype}
      mask prompts: eventid "Identifier of a diagnostic event (EventId)"; DemDebounceBehavior1 "Dem Debounce Behavior 1"; DemDebounceBehavior2 "Dem Debounce Behavior 2"; DemCounterIncrementStepSize "Dem Debounce Counter Increment Step Size"; DemCounterJumpUp "Dem Debounce Counter Jump Up"; DemCounterJumpUpValue "Dem Debounce Counter Jump Up Value"; DemCounterDecrementStepSize "Dem Debounce Counter Decrement Step Size"; DemCounterJumpDown "Dem Debounce Counter Jump Down"; DemCounterJumpDownValue "Dem Debounce Counter Jump Down Value"; DemCounterBypassFailure "Dem Debounce Counter Bypass Failure"
      mask help:
      | It  transmit the status Failed or Passed to the DEM. Accordingly, some bits of the UDS DTC status byte changes synchronously or asynchronously according to the configuration. Debounce is based on counter.
      |
      | -INPUTS-
      | conditionfulfilled: specifies whether the storage condition assigned to the StorageConditionID is fulfilled
      | prefailed: Monitor reports nonqualified test result pre-failed
      | prepassed: Monitor reports nonqualified test result pre-passed
      | failedthreshold: Defines the value of the internal debounce counter, which indicates the failed status.
      | passedthreshold: Defines the value of the internal debounce counter, which indicates the passed status.
      | reseteventdebounce: Freeze or reset the internal debounce counter/timer.
      |
      | -OUTPUTS-
      | debouncevalue: Value of the debounce counter
      | failed: Diagnostic monitor reports an event Failed
      | passed: Diagnostic monitor reports an event passed
      |
      | -PARAMETERS-
      | EventID: Internal identifier of a diagnostic event. 0 is not a valid value.
      | Dem Debounce Behavior: The event debounce counter will be frozen or reset (0 for FREEZE and 1 for RESET)
      | Dem Debounce Counter Increment Step Size: Defines the incrementation  step size for counter (PREFAILED)
      | Dem Debounce Counter Jump Up: Activation of Jump-Up. True: activated. False: deactivated
      | Dem Debounce Counter Jump Up Value: Initialization value for the counter when PREFAILED
      | Dem Debounce Counter Decrement Step Size: Defines the decrementation step for of counter (PREPASSED).
      | Dem Debounce Counter Jump Down: Activation of Jump-Down. True: Jump-Down activated
      | Dem Debounce Counter Jump Down Value: Initialization value for the counter when PREPASSED
      mask init:
      | ThisBlk =gcb;
      | DemDebounceBehaviors = {DemDebounceBehavior1,DemDebounceBehavior2};
      | behaviorblk = [ThisBlk,'/DemDebounceBehavior'];
      | behaviorvector = '[';
      | for cnt=1:2
      |     cnt_str=num2str(cnt);
      |     Bpath = [ThisBlk,'/AEMS_DEM_COUNTER_BASED_DEBOUNCE_THRSHOLD_DYN_CALL',cnt_str,'/AEMS_DEM_COUNTERBASEDDEBOUNCE'];
      | %     set_param(Bpath,'eventid',[eventid,'_' cnt_str]);
      |     if (cnt==1)
      |         set_param(Bpath,'eventid',eventid);
      |     else
      |         Splitname=regexp(eventid,'_','all');
      |         New_EventId=insertBefore(eventid,Splitname(end),num2str(cnt));
      |         set_param(Bpath,'eventid',New_EventId);
      |     end
      |     if strcmpi(DemDebounceBehaviors{cnt},'DEM_DEBOUNCE_FREEZE (0)')
      |         behaviorvector= [behaviorvector,'0,'];
      |     else
      |         behaviorvector= [behaviorvector,'1,'];
      |     end
      | end
      | behaviorvector = behaviorvector(1:end-1);%Why end-1? I want to skip ',' for the last field.
      | behaviorvector = [behaviorvector,']'];
      | set_param(behaviorblk,'Value',behaviorvector);
      settings: AttributesFormatString=|
      | %<MaskType>\nEventId: %<eventid>
      | Dem Debounce Behavior 1 = %<DemDebounceBehavior1>
      | Dem Debounce Behavior 2 = %<DemDebounceBehavior2>
      | Dem Debounce Counter Increment Step Size = %<DemCounterIncrementStepSize>
      | Dem Debounce Counter Jump Up = %<DemCounterJumpUp>
      | Dem Debounce Counter Jump Up Value = %<DemCounterJumpUpValue>
      | Dem Debounce Counter Decrement Step Size = %<DemCounterDecrementStepSize>
      | Dem Debounce Counter Jump Down = %<DemCounterJumpDown>
      | Dem Debounce Counter Jump Down Value = %<DemCounterJumpDownValue>
      | Dem Debounce Counter Bypass Failure = %<DemCounterBypassFailure>
      mask Help:
      | eval('path_lib=fileparts(which(''AEMS_Standard_Library''));');
      | doc_path = [path_lib '\help\AEMS_DEM_COUNTER_BASED_DEBOUNCE_THRSHOLD_DYN.pdf'];
      | eval('open(doc_path)')
      mask TypeOptions DemDebounceBehavior1: DEM_DEBOUNCE_FREEZE (0) | DEM_DEBOUNCE_RESET (1)
      mask TypeOptions DemDebounceBehavior2: DEM_DEBOUNCE_FREEZE (0) | DEM_DEBOUNCE_RESET (1)
  AEMS_DEM_COUNTER_BASED_DEBOUNCE_THRSHOLD_DYN_3D : Subsystem  Tag=[LIB]  Description=This subsystem is interface for self diagnosis standard calculated from similar condition and NG judgment.  mask(AEMS_DEM_COUNTER_BASED_DEBOUNCE_THRSHOLD_DYN_3D){eventid=Dem_EventId_Device_Faulttype, DemDebounceBehavior1=DEM_DEBOUNCE_FREEZE (0), DemDebounceBehavior2=DEM_DEBOUNCE_FREEZE (0), DemDebounceBehavior3=DEM_DEBOUNCE_FREEZE (0), DemCounterIncrementStepSize=Cnx_dem_pfail_inc_step_Device_Faulttype, DemCounterJumpUp=Cbx_dem_jmp_up_act_Device_Faulttype, DemCounterJumpUpValue=Cnx_dem_jmp_up_pfail_Device_Faulttype, DemCounterDecrementStepSize=Cnx_dem_ppass_dec_step_Device_Faulttype, DemCounterJumpDown=Cbx_dem_jmp_dwn_act_Device_Faulttype, DemCounterJumpDownValue=Cnx_dem_jmp_dwn_ppass_Device_Faulttype, DemCounterBypassFailure=Cbx_dem_byp_fail_Device_Faulttype}
      mask prompts: eventid "Identifier of a diagnostic event (EventId)"; DemDebounceBehavior1 "Dem Debounce Behavior 1"; DemDebounceBehavior2 "Dem Debounce Behavior 2"; DemDebounceBehavior3 "Dem Debounce Behavior 3"; DemCounterIncrementStepSize "Dem Debounce Counter Increment Step Size"; DemCounterJumpUp "Dem Debounce Counter Jump Up"; DemCounterJumpUpValue "Dem Debounce Counter Jump Up Value"; DemCounterDecrementStepSize "Dem Debounce Counter Decrement Step Size"; DemCounterJumpDown "Dem Debounce Counter Jump Down"; DemCounterJumpDownValue "Dem Debounce Counter Jump Down Value"; DemCounterBypassFailure "Dem Debounce Counter Bypass Failure"
      mask help:
      | It  transmit the status Failed or Passed to the DEM. Accordingly, some bits of the UDS DTC status byte changes synchronously or asynchronously according to the configuration. Debounce is based on counter.
      |
      | -INPUTS-
      | conditionfulfilled: specifies whether the storage condition assigned to the StorageConditionID is fulfilled
      | prefailed: Monitor reports nonqualified test result pre-failed
      | prepassed: Monitor reports nonqualified test result pre-passed
      | failedthreshold: Defines the value of the internal debounce counter, which indicates the failed status.
      | passedthreshold: Defines the value of the internal debounce counter, which indicates the passed status.
      | reseteventdebounce: Freeze or reset the internal debounce counter/timer.
      |
      | -OUTPUTS-
      | debouncevalue: Value of the debounce counter
      | failed: Diagnostic monitor reports an event Failed
      | passed: Diagnostic monitor reports an event passed
      |
      | -PARAMETERS-
      | EventID: Internal identifier of a diagnostic event. 0 is not a valid value.
      | Dem Debounce Behavior: The event debounce counter will be frozen or reset (0 for FREEZE and 1 for RESET)
      | Dem Debounce Counter Increment Step Size: Defines the incrementation  step size for counter (PREFAILED)
      | Dem Debounce Counter Jump Up: Activation of Jump-Up. True: activated. False: deactivated
      | Dem Debounce Counter Jump Up Value: Initialization value for the counter when PREFAILED
      | Dem Debounce Counter Decrement Step Size: Defines the decrementation step for of counter (PREPASSED).
      | Dem Debounce Counter Jump Down: Activation of Jump-Down. True: Jump-Down activated
      | Dem Debounce Counter Jump Down Value: Initialization value for the counter when PREPASSED
      mask init:
      | ThisBlk =gcb;
      | DemDebounceBehaviors = {DemDebounceBehavior1,DemDebounceBehavior2,DemDebounceBehavior3};   
      | behaviorblk = [ThisBlk,'/DemDebounceBehavior'];
      | behaviorvector = '[';
      |     for cnt=1:3        
      |         cnt_str=num2str(cnt);
      |         Bpath = [ThisBlk,'/AEMS_DEM_COUNTER_BASED_DEBOUNCE_THRSHOLD_DYN_CALL',cnt_str,'/AEMS_DEM_COUNTERBASEDDEBOUNCE'];
      |         %         set_param(Bpath,'eventid',[eventid,'_' cnt_str]);
      |         if (cnt==1)
      |             set_param(Bpath,'eventid',eventid);
      |         else
      |             Splitname=regexp(eventid,'_','all');
      |             New_EventId=insertBefore(eventid,Splitname(end),num2str(cnt));
      |             set_param(Bpath,'eventid',New_EventId);
      |         end
      |         if strcmpi(DemDebounceBehaviors{cnt},'DEM_DEBOUNCE_FREEZE (0)')
      |            behaviorvector= [behaviorvector,'0,'];
      |         else    
      |            behaviorvector= [behaviorvector,'1,'];        
      |         end
      |     end
      |     behaviorvector = behaviorvector(1:end-1);%Why end-1? I want to skip ',' for the last field.
      |     behaviorvector = [behaviorvector,']'];
      |     set_param(behaviorblk,'Value',behaviorvector);
      settings: AttributesFormatString=|
      | %<MaskType>\nEventId: %<eventid>
      | Dem Debounce Behavior 1 = %<DemDebounceBehavior1>
      | Dem Debounce Behavior 2 = %<DemDebounceBehavior2>
      | Dem Debounce Behavior 3 = %<DemDebounceBehavior3>
      | Dem Debounce Counter Increment Step Size = %<DemCounterIncrementStepSize>
      | Dem Debounce Counter Jump Up = %<DemCounterJumpUp>
      | Dem Debounce Counter Jump Up Value = %<DemCounterJumpUpValue>
      | Dem Debounce Counter Decrement Step Size = %<DemCounterDecrementStepSize>
      | Dem Debounce Counter Jump Down = %<DemCounterJumpDown>
      | Dem Debounce Counter Jump Down Value = %<DemCounterJumpDownValue>
      | Dem Debounce Counter Bypass Failure = %<DemCounterBypassFailure>
      mask Help:
      | eval('path_lib=fileparts(which(''AEMS_Standard_Library''));');
      | doc_path = [path_lib '\help\AEMS_DEM_COUNTER_BASED_DEBOUNCE_THRSHOLD_DYN.pdf'];
      | eval('open(doc_path)')
      mask TypeOptions DemDebounceBehavior1: DEM_DEBOUNCE_FREEZE (0) | DEM_DEBOUNCE_RESET (1)
      mask TypeOptions DemDebounceBehavior2: DEM_DEBOUNCE_FREEZE (0) | DEM_DEBOUNCE_RESET (1)
      mask TypeOptions DemDebounceBehavior3: DEM_DEBOUNCE_FREEZE (0) | DEM_DEBOUNCE_RESET (1)
  AEMS_DEM_COUNTER_BASED_DEBOUNCE_THRSHOLD_DYN_4D : Subsystem  Tag=[LIB]  Description=This subsystem is interface for self diagnosis standard calculated from similar condition and NG judgment.  mask(AEMS_DEM_COUNTER_BASED_DEBOUNCE_THRSHOLD_DYN_4D){eventid=Dem_EventId_Device_Faulttype, DemDebounceBehavior1=DEM_DEBOUNCE_FREEZE (0), DemDebounceBehavior2=DEM_DEBOUNCE_FREEZE (0), DemDebounceBehavior3=DEM_DEBOUNCE_FREEZE (0), DemDebounceBehavior4=DEM_DEBOUNCE_FREEZE (0), DemCounterIncrementStepSize=Cnx_dem_pfail_inc_step_Device_Faulttype, DemCounterJumpUp=Cbx_dem_jmp_up_act_Device_Faulttype, DemCounterJumpUpValue=Cnx_dem_jmp_up_pfail_Device_Faulttype, DemCounterDecrementStepSize=Cnx_dem_ppass_dec_step_Device_Faulttype, DemCounterJumpDown=Cbx_dem_jmp_dwn_act_Device_Faulttype, DemCounterJumpDownValue=Cnx_dem_jmp_dwn_ppass_Device_Faulttype, DemCounterBypassFailure=Cbx_dem_byp_fail_Device_Faulttype}
      mask prompts: eventid "Identifier of a diagnostic event (EventId)"; DemDebounceBehavior1 "Dem Debounce Behavior 1"; DemDebounceBehavior2 "Dem Debounce Behavior 2"; DemDebounceBehavior3 "Dem Debounce Behavior 3"; DemDebounceBehavior4 "Dem Debounce Behavior 4"; DemCounterIncrementStepSize "Dem Debounce Counter Increment Step Size"; DemCounterJumpUp "Dem Debounce Counter Jump Up"; DemCounterJumpUpValue "Dem Debounce Counter Jump Up Value"; DemCounterDecrementStepSize "Dem Debounce Counter Decrement Step Size"; DemCounterJumpDown "Dem Debounce Counter Jump Down"; DemCounterJumpDownValue "Dem Debounce Counter Jump Down Value"; DemCounterBypassFailure "Dem Debounce Counter Bypass Failure"
      mask help:
      | It  transmit the status Failed or Passed to the DEM. Accordingly, some bits of the UDS DTC status byte changes synchronously or asynchronously according to the configuration. Debounce is based on counter.
      |
      | -INPUTS-
      | conditionfulfilled: specifies whether the storage condition assigned to the StorageConditionID is fulfilled
      | prefailed: Monitor reports nonqualified test result pre-failed
      | prepassed: Monitor reports nonqualified test result pre-passed
      | failedthreshold: Defines the value of the internal debounce counter, which indicates the failed status.
      | passedthreshold: Defines the value of the internal debounce counter, which indicates the passed status.
      | reseteventdebounce: Freeze or reset the internal debounce counter/timer.
      |
      | -OUTPUTS-
      | debouncevalue: Value of the debounce counter
      | failed: Diagnostic monitor reports an event Failed
      | passed: Diagnostic monitor reports an event passed
      |
      | -PARAMETERS-
      | EventID: Internal identifier of a diagnostic event. 0 is not a valid value.
      | Dem Debounce Behavior: The event debounce counter will be frozen or reset (0 for FREEZE and 1 for RESET)
      | Dem Debounce Counter Increment Step Size: Defines the incrementation  step size for counter (PREFAILED)
      | Dem Debounce Counter Jump Up: Activation of Jump-Up. True: activated. False: deactivated
      | Dem Debounce Counter Jump Up Value: Initialization value for the counter when PREFAILED
      | Dem Debounce Counter Decrement Step Size: Defines the decrementation step for of counter (PREPASSED).
      | Dem Debounce Counter Jump Down: Activation of Jump-Down. True: Jump-Down activated
      | Dem Debounce Counter Jump Down Value: Initialization value for the counter when PREPASSED
      mask init:
      | ThisBlk =gcb;
      | DemDebounceBehaviors = {DemDebounceBehavior1,DemDebounceBehavior2,DemDebounceBehavior3,DemDebounceBehavior4};   
      | behaviorblk = [ThisBlk,'/DemDebounceBehavior'];
      | behaviorvector = '[';
      |     for cnt=1:4        
      |         cnt_str=num2str(cnt);
      |         Bpath = [ThisBlk,'/AEMS_DEM_COUNTER_BASED_DEBOUNCE_THRSHOLD_DYN_CALL',cnt_str,'/AEMS_DEM_COUNTERBASEDDEBOUNCE'];
      |         %         set_param(Bpath,'eventid',[eventid,'_' cnt_str]);
      |         if (cnt==1)
      |             set_param(Bpath,'eventid',eventid);
      |         else
      |             Splitname=regexp(eventid,'_','all');
      |             New_EventId=insertBefore(eventid,Splitname(end),num2str(cnt));
      |             set_param(Bpath,'eventid',New_EventId);
      |         end
      |         if strcmpi(DemDebounceBehaviors{cnt},'DEM_DEBOUNCE_FREEZE (0)')
      |            behaviorvector= [behaviorvector,'0,'];
      |         else    
      |            behaviorvector= [behaviorvector,'1,'];        
      |         end
      |     end
      |     behaviorvector = behaviorvector(1:end-1);%Why end-1? I want to skip ',' for the last field.
      |     behaviorvector = [behaviorvector,']'];
      |     set_param(behaviorblk,'Value',behaviorvector);
      settings: AttributesFormatString=|
      | %<MaskType>\nEventId: %<eventid>
      | Dem Debounce Behavior 1 = %<DemDebounceBehavior1>
      | Dem Debounce Behavior 2 = %<DemDebounceBehavior2>
      | Dem Debounce Behavior 3 = %<DemDebounceBehavior3>
      | Dem Debounce Behavior 4 = %<DemDebounceBehavior4>
      | Dem Debounce Counter Increment Step Size = %<DemCounterIncrementStepSize>
      | Dem Debounce Counter Jump Up = %<DemCounterJumpUp>
      | Dem Debounce Counter Jump Up Value = %<DemCounterJumpUpValue>
      | Dem Debounce Counter Decrement Step Size = %<DemCounterDecrementStepSize>
      | Dem Debounce Counter Jump Down = %<DemCounterJumpDown>
      | Dem Debounce Counter Jump Down Value = %<DemCounterJumpDownValue>
      | Dem Debounce Counter Bypass Failure = %<DemCounterBypassFailure>
      mask Help:
      | eval('path_lib=fileparts(which(''AEMS_Standard_Library''));');
      | doc_path = [path_lib '\help\AEMS_DEM_COUNTER_BASED_DEBOUNCE_THRSHOLD_DYN.pdf'];
      | eval('open(doc_path)')
      mask TypeOptions DemDebounceBehavior1: DEM_DEBOUNCE_FREEZE (0) | DEM_DEBOUNCE_RESET (1)
      mask TypeOptions DemDebounceBehavior2: DEM_DEBOUNCE_FREEZE (0) | DEM_DEBOUNCE_RESET (1)
      mask TypeOptions DemDebounceBehavior3: DEM_DEBOUNCE_FREEZE (0) | DEM_DEBOUNCE_RESET (1)
      mask TypeOptions DemDebounceBehavior4: DEM_DEBOUNCE_FREEZE (0) | DEM_DEBOUNCE_RESET (1)
  AEMS_DEM_COUNTER_BASED_DEBOUNCE_THRSHOLD_DYN_6D : Subsystem  Tag=[LIB]  Description=This subsystem is interface for self diagnosis standard calculated from similar condition and NG judgment.  mask(AEMS_DEM_COUNTER_BASED_DEBOUNCE_THRSHOLD_DYN_6D){eventid=Dem_EventId_Device_Faulttype, DemDebounceBehavior1=DEM_DEBOUNCE_FREEZE (0), DemDebounceBehavior2=DEM_DEBOUNCE_FREEZE (0), DemDebounceBehavior3=DEM_DEBOUNCE_FREEZE (0), DemDebounceBehavior4=DEM_DEBOUNCE_FREEZE (0), DemDebounceBehavior5=DEM_DEBOUNCE_FREEZE (0), DemDebounceBehavior6=DEM_DEBOUNCE_FREEZE (0), DemCounterIncrementStepSize=Cnx_dem_pfail_inc_step_Device_Faulttype, DemCounterJumpUp=Cbx_dem_jmp_up_act_Device_Faulttype, DemCounterJumpUpValue=Cnx_dem_jmp_up_pfail_Device_Faulttype, DemCounterDecrementStepSize=Cnx_dem_ppass_dec_step_Device_Faulttype, DemCounterJumpDown=Cbx_dem_jmp_dwn_act_Device_Faulttype, DemCounterJumpDownValue=Cnx_dem_jmp_dwn_ppass_Device_Faulttype, DemCounterBypassFailure=Cbx_dem_byp_fail_Device_Faulttype}
      mask prompts: eventid "Identifier of a diagnostic event (EventId)"; DemDebounceBehavior1 "Dem Debounce Behavior 1"; DemDebounceBehavior2 "Dem Debounce Behavior 2"; DemDebounceBehavior3 "Dem Debounce Behavior 3"; DemDebounceBehavior4 "Dem Debounce Behavior 4"; DemDebounceBehavior5 "Dem Debounce Behavior 5"; DemDebounceBehavior6 "Dem Debounce Behavior 6"; DemCounterIncrementStepSize "Dem Debounce Counter Increment Step Size"; DemCounterJumpUp "Dem Debounce Counter Jump Up"; DemCounterJumpUpValue "Dem Debounce Counter Jump Up Value"; DemCounterDecrementStepSize "Dem Debounce Counter Decrement Step Size"; DemCounterJumpDown "Dem Debounce Counter Jump Down"; DemCounterJumpDownValue "Dem Debounce Counter Jump Down Value"; DemCounterBypassFailure "Dem Debounce Counter Bypass Failure"
      mask help:
      | It  transmit the status Failed or Passed to the DEM. Accordingly, some bits of the UDS DTC status byte changes synchronously or asynchronously according to the configuration. Debounce is based on counter.
      |
      | -INPUTS-
      | conditionfulfilled: specifies whether the storage condition assigned to the StorageConditionID is fulfilled
      | prefailed: Monitor reports nonqualified test result pre-failed
      | prepassed: Monitor reports nonqualified test result pre-passed
      | failedthreshold: Defines the value of the internal debounce counter, which indicates the failed status.
      | passedthreshold: Defines the value of the internal debounce counter, which indicates the passed status.
      | reseteventdebounce: Freeze or reset the internal debounce counter/timer.
      |
      | -OUTPUTS-
      | debouncevalue: Value of the debounce counter
      | failed: Diagnostic monitor reports an event Failed
      | passed: Diagnostic monitor reports an event passed
      |
      | -PARAMETERS-
      | EventID: Internal identifier of a diagnostic event. 0 is not a valid value.
      | Dem Debounce Behavior: The event debounce counter will be frozen or reset (0 for FREEZE and 1 for RESET)
      | Dem Debounce Counter Increment Step Size: Defines the incrementation  step size for counter (PREFAILED)
      | Dem Debounce Counter Jump Up: Activation of Jump-Up. True: activated. False: deactivated
      | Dem Debounce Counter Jump Up Value: Initialization value for the counter when PREFAILED
      | Dem Debounce Counter Decrement Step Size: Defines the decrementation step for of counter (PREPASSED).
      | Dem Debounce Counter Jump Down: Activation of Jump-Down. True: Jump-Down activated
      | Dem Debounce Counter Jump Down Value: Initialization value for the counter when PREPASSED
      mask init:
      | ThisBlk =gcb;
      | DemDebounceBehaviors = {DemDebounceBehavior1,DemDebounceBehavior2,DemDebounceBehavior3,DemDebounceBehavior4,DemDebounceBehavior5,DemDebounceBehavior6};   
      | behaviorblk = [ThisBlk,'/DemDebounceBehavior'];
      | behaviorvector = '[';
      |     for cnt=1:6        
      |         cnt_str=num2str(cnt);
      |         Bpath = [ThisBlk,'/AEMS_DEM_COUNTER_BASED_DEBOUNCE_THRSHOLD_DYN_CALL',cnt_str,'/AEMS_DEM_COUNTERBASEDDEBOUNCE'];
      | %         set_param(Bpath,'eventid',[eventid,'_' cnt_str]);
      |         if (cnt==1)
      |             set_param(Bpath,'eventid',eventid);
      |         else
      |             Splitname=regexp(eventid,'_','all');
      |             New_EventId=insertBefore(eventid,Splitname(end),num2str(cnt));
      |             set_param(Bpath,'eventid',New_EventId);
      |         end
      |         if strcmpi(DemDebounceBehaviors{cnt},'DEM_DEBOUNCE_FREEZE (0)')
      |            behaviorvector= [behaviorvector,'0,'];
      |         else    
      |            behaviorvector= [behaviorvector,'1,'];        
      |         end
      |     end
      |     behaviorvector = behaviorvector(1:end-1);%Why end-1? I want to skip ',' for the last field.
      |     behaviorvector = [behaviorvector,']'];
      |     set_param(behaviorblk,'Value',behaviorvector);
      settings: AttributesFormatString=|
      | %<MaskType>\nEventId: %<eventid>
      | Dem Debounce Behavior 1 = %<DemDebounceBehavior1>
      | Dem Debounce Behavior 2 = %<DemDebounceBehavior2>
      | Dem Debounce Behavior 3 = %<DemDebounceBehavior3>
      | Dem Debounce Behavior 4 = %<DemDebounceBehavior4>
      | Dem Debounce Behavior 5 = %<DemDebounceBehavior5>
      | Dem Debounce Behavior 6 = %<DemDebounceBehavior6>
      | Dem Debounce Counter Increment Step Size = %<DemCounterIncrementStepSize>
      | Dem Debounce Counter Jump Up = %<DemCounterJumpUp>
      | Dem Debounce Counter Jump Up Value = %<DemCounterJumpUpValue>
      | Dem Debounce Counter Decrement Step Size = %<DemCounterDecrementStepSize>
      | Dem Debounce Counter Jump Down = %<DemCounterJumpDown>
      | Dem Debounce Counter Jump Down Value = %<DemCounterJumpDownValue>
      | Dem Debounce Counter Bypass Failure = %<DemCounterBypassFailure>
      mask Help:
      | eval('path_lib=fileparts(which(''AEMS_Standard_Library''));');
      | doc_path = [path_lib '\help\AEMS_DEM_COUNTER_BASED_DEBOUNCE_THRSHOLD_DYN.pdf'];
      | eval('open(doc_path)')
      mask TypeOptions DemDebounceBehavior1: DEM_DEBOUNCE_FREEZE (0) | DEM_DEBOUNCE_RESET (1)
      mask TypeOptions DemDebounceBehavior2: DEM_DEBOUNCE_FREEZE (0) | DEM_DEBOUNCE_RESET (1)
      mask TypeOptions DemDebounceBehavior3: DEM_DEBOUNCE_FREEZE (0) | DEM_DEBOUNCE_RESET (1)
      mask TypeOptions DemDebounceBehavior4: DEM_DEBOUNCE_FREEZE (0) | DEM_DEBOUNCE_RESET (1)
      mask TypeOptions DemDebounceBehavior5: DEM_DEBOUNCE_FREEZE (0) | DEM_DEBOUNCE_RESET (1)
      mask TypeOptions DemDebounceBehavior6: DEM_DEBOUNCE_FREEZE (0) | DEM_DEBOUNCE_RESET (1)
  AEMS_DEM_COUNTER_BASED_DEBOUNCE_THRSHOLD_DYN_8D : Subsystem  Tag=[LIB]  Description=This subsystem is interface for self diagnosis standard calculated from similar condition and NG judgment.  mask(AEMS_DEM_COUNTER_BASED_DEBOUNCE_THRSHOLD_DYN_8D){eventid=Dem_EventId_Device_Faulttype, DemDebounceBehavior1=DEM_DEBOUNCE_FREEZE (0), DemDebounceBehavior2=DEM_DEBOUNCE_FREEZE (0), DemDebounceBehavior3=DEM_DEBOUNCE_FREEZE (0), DemDebounceBehavior4=DEM_DEBOUNCE_FREEZE (0), DemDebounceBehavior5=DEM_DEBOUNCE_FREEZE (0), DemDebounceBehavior6=DEM_DEBOUNCE_FREEZE (0), DemDebounceBehavior7=DEM_DEBOUNCE_FREEZE (0), DemDebounceBehavior8=DEM_DEBOUNCE_FREEZE (0), DemCounterIncrementStepSize=Cnx_dem_pfail_inc_step_Device_Faulttype, DemCounterJumpUp=Cbx_dem_jmp_up_act_Device_Faulttype, DemCounterJumpUpValue=Cnx_dem_jmp_up_pfail_Device_Faulttype, DemCounterDecrementStepSize=Cnx_dem_ppass_dec_step_Device_Faulttype, DemCounterJumpDown=Cbx_dem_jmp_dwn_act_Device_Faulttype, DemCounterJumpDownValue=Cnx_dem_jmp_dwn_ppass_Device_Faulttype, DemCounterBypassFailure=Cbx_dem_byp_fail_Device_Faulttype}
      mask prompts: eventid "Identifier of a diagnostic event (EventId)"; DemDebounceBehavior1 "Dem Debounce Behavior 1"; DemDebounceBehavior2 "Dem Debounce Behavior 2"; DemDebounceBehavior3 "Dem Debounce Behavior 3"; DemDebounceBehavior4 "Dem Debounce Behavior 4"; DemDebounceBehavior5 "Dem Debounce Behavior 5"; DemDebounceBehavior6 "Dem Debounce Behavior 6"; DemDebounceBehavior7 "Dem Debounce Behavior 7"; DemDebounceBehavior8 "Dem Debounce Behavior 8"; DemCounterIncrementStepSize "Dem Debounce Counter Increment Step Size"; DemCounterJumpUp "Dem Debounce Counter Jump Up"; DemCounterJumpUpValue "Dem Debounce Counter Jump Up Value"; DemCounterDecrementStepSize "Dem Debounce Counter Decrement Step Size"; DemCounterJumpDown "Dem Debounce Counter Jump Down"; DemCounterJumpDownValue "Dem Debounce Counter Jump Down Value"; DemCounterBypassFailure "Dem Debounce Counter Bypass Failure"
      mask help:
      | It  transmit the status Failed or Passed to the DEM. Accordingly, some bits of the UDS DTC status byte changes synchronously or asynchronously according to the configuration. Debounce is based on counter.
      |
      | -INPUTS-
      | conditionfulfilled: specifies whether the storage condition assigned to the StorageConditionID is fulfilled
      | prefailed: Monitor reports nonqualified test result pre-failed
      | prepassed: Monitor reports nonqualified test result pre-passed
      | failedthreshold: Defines the value of the internal debounce counter, which indicates the failed status.
      | passedthreshold: Defines the value of the internal debounce counter, which indicates the passed status.
      | reseteventdebounce: Freeze or reset the internal debounce counter/timer.
      |
      | -OUTPUTS-
      | debouncevalue: Value of the debounce counter
      | failed: Diagnostic monitor reports an event Failed
      | passed: Diagnostic monitor reports an event passed
      |
      | -PARAMETERS-
      | EventID: Internal identifier of a diagnostic event. 0 is not a valid value.
      | Dem Debounce Behavior: The event debounce counter will be frozen or reset (0 for FREEZE and 1 for RESET)
      | Dem Debounce Counter Increment Step Size: Defines the incrementation  step size for counter (PREFAILED)
      | Dem Debounce Counter Jump Up: Activation of Jump-Up. True: activated. False: deactivated
      | Dem Debounce Counter Jump Up Value: Initialization value for the counter when PREFAILED
      | Dem Debounce Counter Decrement Step Size: Defines the decrementation step for of counter (PREPASSED).
      | Dem Debounce Counter Jump Down: Activation of Jump-Down. True: Jump-Down activated
      | Dem Debounce Counter Jump Down Value: Initialization value for the counter when PREPASSED
      mask init:
      | ThisBlk =gcb;
      | DemDebounceBehaviors = {DemDebounceBehavior1,DemDebounceBehavior2,DemDebounceBehavior3,DemDebounceBehavior4,DemDebounceBehavior5,DemDebounceBehavior6,DemDebounceBehavior7,DemDebounceBehavior8};   
      | behaviorblk = [ThisBlk,'/DemDebounceBehavior'];
      | behaviorvector = '[';
      |     for cnt=1:8        
      |         cnt_str=num2str(cnt);
      |         Bpath = [ThisBlk,'/AEMS_DEM_COUNTER_BASED_DEBOUNCE_THRSHOLD_DYN_CALL',cnt_str,'/AEMS_DEM_COUNTERBASEDDEBOUNCE'];
      | %         set_param(Bpath,'eventid',[eventid,'_' cnt_str]);
      |         if (cnt==1)
      |             set_param(Bpath,'eventid',eventid);
      |         else
      |             Splitname=regexp(eventid,'_','all');
      |             New_EventId=insertBefore(eventid,Splitname(end),num2str(cnt));
      |             set_param(Bpath,'eventid',New_EventId);
      |         end
      |         if strcmpi(DemDebounceBehaviors{cnt},'DEM_DEBOUNCE_FREEZE (0)')
      |            behaviorvector= [behaviorvector,'0,'];
      |         else    
      |            behaviorvector= [behaviorvector,'1,'];        
      |         end
      |     end
      |     behaviorvector = behaviorvector(1:end-1);%Why end-1? I want to skip ',' for the last field.
      |     behaviorvector = [behaviorvector,']'];
      |     set_param(behaviorblk,'Value',behaviorvector);
      settings: AttributesFormatString=|
      | %<MaskType>\nEventId: %<eventid>
      | Dem Debounce Behavior 1 = %<DemDebounceBehavior1>
      | Dem Debounce Behavior 2 = %<DemDebounceBehavior2>
      | Dem Debounce Behavior 3 = %<DemDebounceBehavior3>
      | Dem Debounce Behavior 4 = %<DemDebounceBehavior4>
      | Dem Debounce Behavior 5 = %<DemDebounceBehavior5>
      | Dem Debounce Behavior 6 = %<DemDebounceBehavior6>
      | Dem Debounce Behavior 7 = %<DemDebounceBehavior7>
      | Dem Debounce Behavior 8 = %<DemDebounceBehavior8>
      | Dem Debounce Counter Increment Step Size = %<DemCounterIncrementStepSize>
      | Dem Debounce Counter Jump Up = %<DemCounterJumpUp>
      | Dem Debounce Counter Jump Up Value = %<DemCounterJumpUpValue>
      | Dem Debounce Counter Decrement Step Size = %<DemCounterDecrementStepSize>
      | Dem Debounce Counter Jump Down = %<DemCounterJumpDown>
      | Dem Debounce Counter Jump Down Value = %<DemCounterJumpDownValue>
      | Dem Debounce Counter Bypass Failure = %<DemCounterBypassFailure>
      mask Help:
      | eval('path_lib=fileparts(which(''AEMS_Standard_Library''));');
      | doc_path = [path_lib '\help\AEMS_DEM_COUNTER_BASED_DEBOUNCE_THRSHOLD_DYN.pdf'];
      | eval('open(doc_path)')
      mask TypeOptions DemDebounceBehavior1: DEM_DEBOUNCE_FREEZE (0) | DEM_DEBOUNCE_RESET (1)
      mask TypeOptions DemDebounceBehavior2: DEM_DEBOUNCE_FREEZE (0) | DEM_DEBOUNCE_RESET (1)
      mask TypeOptions DemDebounceBehavior3: DEM_DEBOUNCE_FREEZE (0) | DEM_DEBOUNCE_RESET (1)
      mask TypeOptions DemDebounceBehavior4: DEM_DEBOUNCE_FREEZE (0) | DEM_DEBOUNCE_RESET (1)
      mask TypeOptions DemDebounceBehavior5: DEM_DEBOUNCE_FREEZE (0) | DEM_DEBOUNCE_RESET (1)
      mask TypeOptions DemDebounceBehavior6: DEM_DEBOUNCE_FREEZE (0) | DEM_DEBOUNCE_RESET (1)
      mask TypeOptions DemDebounceBehavior7: DEM_DEBOUNCE_FREEZE (0) | DEM_DEBOUNCE_RESET (1)
      mask TypeOptions DemDebounceBehavior8: DEM_DEBOUNCE_FREEZE (0) | DEM_DEBOUNCE_RESET (1)
  AEMS_DEM_GETEVENTSTATUS : Subsystem  Tag=[LIB]  mask(AEMS_DEM_GETEVENTSTATUS){EventId=EventId_XXXX, FunctionMode=Dysfunctional}
      mask prompts: EventId "EventId :"; FunctionMode "Function Mode"
      mask help:
      | This library calls AUTOSAR standard functions.
      | Refer the AUTOSAR Dem_GetEventStatus [SWS_Dem_00195]
      mask init:
      | Thisblk = gcb;
      | Src_Of_Permission_Port = [Thisblk,'/Source_Of_Permission_Port'];
      | BlkType_Of_Source_Of_Permission_Port  = get_param(Src_Of_Permission_Port ,'BlockType');
      | 
      | if strcmp(FunctionMode,'Dysfunctional')
      |     if strcmp(BlkType_Of_Source_Of_Permission_Port  ,'Ground')
      |         %do nothing
      |     else
      |         replace_block(Src_Of_Permission_Port,'FollowLinks','on','BlockType','DataStoreRead','Ground','noprompt');
      |     end        
      |     
      | elseif strcmp(FunctionMode,'From Data Store memory')
      |     if strcmp(BlkType_Of_Source_Of_Permission_Port  ,'DataStoreRead')
      |         %do nothing
      |     else 
      |         replace_block(Src_Of_Permission_Port,'FollowLinks','on','BlockType','Ground','DataStoreRead','noprompt');
      |     end
      |     
      | model_type_pos = strsplit(Thisblk,'/');%to split all the layer paths in order to get the runnable path
      | runnable_path = [bdroot '/' model_type_pos{2}];%to get the runnable or APICALL path
      | trg_port_name = get_param(find_system(runnable_path,'BlockType','TriggerPort'),'Name');%to get the function call trigger name
      | TaskRate = '';%the raster suffix is stored in the parameter    
      |     
      |     %Get Task Rate of this block.(As per AEMS arch, all the blks shall be
      |     %kept under the runnable. The Runnable name will ncontain the sample
      |     %time suffix. From where we can get it.
      |  if ~isempty(trg_port_name)
      |     trg_port_name_spltd = strsplit(trg_port_name{1},'_');%splitting is done in order to get the raster and its type(Sched or Event)
      |     
      |     % checking for rasters of type Sched or Event especially occuring in
      |     % runnables
      |     if ~isempty(regexp(trg_port_name_spltd{1},'^Sched|^Event','once')) 
      |         TaskRate = ['_' regexprep(trg_port_name_spltd{1},'Sched|Event','','once')];
      |         
      |     %checking if the raster is dcmcb and this is applicable only for
      |     %APICALL
      |     elseif ~isempty(regexp([trg_port_name_spltd{1} '_' trg_port_name_spltd{2} '_' ],'^DataServices_DCM_|^RoutineServices_DCM_','once'))||...
      |             ~isempty(regexp(trg_port_name_spltd{1},'^Dcm$','once'))
      |         TaskRate = '_dcmcb';
      |         
      |     %checking if this block is used under the function call trigger
      |     %starting with "Com" and then giving an error message
      |     %this is applicable only for APICALL
      |     elseif ~isempty(regexp(trg_port_name_spltd{1},'^Com$','once'))
      |         msg = sprintf(['\n','The GETEVENTSTATUS block "' Thisblk '" should not be present within APICALLs having function call trigger as "Com"']);
      |         errordlg(msg);
      |         return;
      |     end
      | end   
      | 
      |     DataStoreName = [EventId,TaskRate];
      | %     Data_Store_Name = get_param([Thisblk,'/Source_Of_Permission_Port'],'DataStoreName');
      | %     if ~isequal(DataStoreName, Data_Store_Name)
      |         set_param([Thisblk,'/Source_Of_Permission_Port'],'DataStoreName',DataStoreName);
      | %     end
      | end
      | % name_show = get_param([Thisblk,'/Source_Of_Permission_Port'],'ShowName');
      | % if isequal(name_show,'on')
      |     set_param([Thisblk,'/Source_Of_Permission_Port'],'ShowName','off');
      | % end
      settings: AttributesFormatString=%<MaskType>\nFunction Mode : = %<FunctionMode>
      mask TypeOptions FunctionMode: Dysfunctional | From Data Store memory
      mask Display:
      | disp(['Dem_GetEventStatus \n \n \n \n \n']);
      | plot([5,5,5])
      | plot([6,6,6])
      | port_label('input',1,'EventId')
      | % port_label('input',2,'dummy')
      | port_label('output',1,'EventStatusExtended')
      | % port_label('output',2,'DemResult')
  AEMS_DEM_GETINDICATORSTATUS : Subsystem  Tag=[LIB]  mask(AEMS_DEM_GETINDICATORSTATUS){IndicatorId=0 : IndicatorOff, SimulationMode=0 : Indicator off mode}
      mask prompts: IndicatorId "IndicatorId :"; SimulationMode "Simulation Mode"
      mask help:
      | This library calls AUTOSAR standard functions.
      | To know more details, please refer AUTOSAR DEM00205.
      mask init:
      | Thisblk = gcb;
      | Src_Of_Permission_Port = [Thisblk,'/Source_Of_Permission_Port'];
      | BlkType_Of_Source_Of_Permission_Port  = get_param(Src_Of_Permission_Port ,'BlockType');
      | 
      | if strcmp(SimulationMode,'From Data Store memory')
      |     if strcmp(BlkType_Of_Source_Of_Permission_Port  ,'DataStoreRead')
      |         %do nothing
      |     else 
      |         replace_block(Src_Of_Permission_Port,'FollowLinks','on','BlockType','Constant','DataStoreRead','noprompt');
      |     end
      | 
      | model_type_pos = strsplit(Thisblk,'/');%to split all the layer paths in order to get the runnable path
      | runnable_path = [bdroot '/' model_type_pos{2}];%to get the runnable or AIPCALL path
      | trg_port_name = get_param(find_system(runnable_path,'BlockType','TriggerPort'),'Name');%to get the function call trigger name
      | TaskRate = '';%the raster suffix is stored in the parameter 
      | 
      | if ~isempty(trg_port_name)
      |     trg_port_name_spltd = strsplit(trg_port_name{1},'_');%splitting is done in order to get the raster and its type(Sched or Event)
      |     
      |     % checking for rasters of type Sched or Event especially occuring in
      |     % runnables
      |     if ~isempty(regexp(trg_port_name_spltd{1},'^Sched\d+(ms|s)$|^Event+(sync|knock|comc|coml|dcmcb)$','once')) 
      |         TaskRate = ['_' regexp(trg_port_name_spltd{1},'\d+(ms|s)$|sync$|knock$|comc$|coml$|dcmcb$','match','once')];
      |         
      |     %checking if the raster is dcmcb and this is applicable only for
      |     %APICALL
      |     elseif ~isempty(regexp([trg_port_name_spltd{1} '_' trg_port_name_spltd{2} '_' ],'^DataServices_DCM_|^RoutineServices_DCM_','once'))||...
      |             ~isempty(regexp(trg_port_name_spltd{1},'^Dcm$','once'))
      |         TaskRate = '_dcmcb';
      |         
      |     %checking if this block is used under the function call trigger
      |     %starting with "Com" and then giving an error message
      |     %this is applicable only for APICALL
      |     elseif ~isempty(regexp(trg_port_name_spltd{1},'^Com$','once'))
      |         msg = sprintf(['\n','The DEM_GETINDICATORSTATUS block "' Thisblk '" should not be present within APICALLs having function call trigger as "Com"']);
      |         errordlg(msg);
      |         return;
      |     end
      | end
      | indicator_label = IndicatorId(strfind(IndicatorId,':')+2:length(IndicatorId));
      | 
      | DataStoreName = [indicator_label TaskRate];%the variable name that should be given to DataStoreRead block 
      | set_param([Thisblk,'/Source_Of_Permission_Port'],'DataStoreName',DataStoreName);
      | 
      | else
      |     replace_block(Src_Of_Permission_Port,'FollowLinks','on','BlockType','DataStoreRead','Constant','noprompt');
      |     set_param([Thisblk,'/Source_Of_Permission_Port'],'OutDataTypeStr','Inherit: Inherit via back propagation');
      |     
      |     if strcmp(SimulationMode,'0 : Indicator off mode')
      |         set_param([Thisblk,'/Source_Of_Permission_Port'],'Value','0');
      |         
      |     elseif strcmp(SimulationMode,'1 : Indicator continuously on mode')
      |         set_param([Thisblk,'/Source_Of_Permission_Port'],'Value','1');
      |         
      |     elseif strcmp(SimulationMode,'2 : Indicator blinking mode')
      |         set_param([Thisblk,'/Source_Of_Permission_Port'],'Value','2');
      |         
      |     elseif strcmp(SimulationMode,'3 : Indicator blinking or continuously on mode')
      |         set_param([Thisblk,'/Source_Of_Permission_Port'],'Value','3');
      |         
      |     elseif strcmp(SimulationMode,'4 : Indicator slow flashing mode')
      |         set_param([Thisblk,'/Source_Of_Permission_Port'],'Value','4');
      |         
      |     elseif strcmp(SimulationMode,'5 : Indicator fast flashing mode')
      |         set_param([Thisblk,'/Source_Of_Permission_Port'],'Value','5');
      |         
      |     elseif strcmp(SimulationMode,'6 : Indicator on-demand mode')
      |         set_param([Thisblk,'/Source_Of_Permission_Port'],'Value','6');
      |         
      |     elseif strcmp(SimulationMode,'7 : Indicator short mode')
      |         set_param([Thisblk,'/Source_Of_Permission_Port'],'Value','7');
      |     end   
      | end
      settings: AttributesFormatString=|
      | %<MaskType>\nIndicatorId = %<IndicatorId>
      | Simulation Mode = %<SimulationMode>
      mask TypeOptions IndicatorId: 0 : IndicatorOff | 1 : DemMILIndicator | 2 : DemRedStopIndicator | 3 : DemAmberWarningIndicator | 4 : DemMessageIndicator1 | 5 : DemMessageIndicator2 | 6 : DemMessageIndicator3 | 7 : DemMessageIndicator4 | 8 : DemMessageIndicator5 | 9 : DemMessageIndicator6 | 10 : DemMessageIndicator7 | 11 : DemMessageIndicator8 | 12 : DemMessageIndicator9 | 13 : DemMessageIndicator10 | 14 : DemMessageIndicator11 | 15 : DemMessageIndicator12 | 16 : DemMessageIndicator13 | 17 : DemMessageIndicator14 | 18 : DemMessageIndicator15 | 19 : DemMessageIndicator16 | 20 : DemMessageIndicator17 | 21 : DemMessageIndicator18 | 22 : DemMessageIndicator19 | 23 : DemMessageIndicator20
      mask TypeOptions SimulationMode: 0 : Indicator off mode | 1 : Indicator continuously on mode | 2 : Indicator blinking mode | 3 : Indicator blinking or continuously on mode | 4 : Indicator slow flashing mode | 5 : Indicator fast flashing mode | 6 : Indicator on-demand mode | 7 : Indicator short mode | From Data Store memory
      mask Display:
      | disp(['Dem_GetIndicatorStatus \n \n \n \n \n']);
      | plot([5,5,5])
      | plot([6,6,6])
      | port_label('input',1,'IndicatorId')
      | port_label('output',1,'IndicatorStatus')
  AEMS_DEM_GET_EVENT_STS_1D : Subsystem  Tag=[LIB]  mask(AEMS_DEM_GET_EVENT_STS_1D){EventId=Dem_EventId_XXX, LibType=_DGN, FunctionMode=Dysfunctional}
      mask prompts: EventId "EventId :"; LibType "DEM Library type :"; FunctionMode "Function Mode"
      mask init:
      | eval([char(EventId) '= 0;'])
      | lib_path = gcb;
      | set_param([lib_path,'/AEMS_DEM_GETEVENTSTATUS'],'EventId',char(EventId));
      | set_param([lib_path,'/AEMS_DEM_GETEVENTSTATUS'],'FunctionMode',FunctionMode);
      | 
      | eventid_b = find_system(lib_path,'LookUnderMasks','all','FollowLinks','on','Name','EventId_Block');
      | set_param([eventid_b{:}],'Value',char(EventId));
      | bit_ext_b = find_system(lib_path,'LookUnderMasks','all','FollowLinks','on','Name','AEMS_DEM_LIB_BIT_EXTRACT');
      | 
      |       
      | 
      | switch LibType
      |     case '_DGN'
      |         if ismember(get_param(bit_ext_b,'MaskType'),{'AEMS_DEM_LIB_BIT_EXTRACT'})
      |         else
      |             replace_block(lib_path,'FollowLinks','on','Name','AEMS_DEM_LIB_BIT_EXTRACT','AEMS_Standard_Library/SUB/AEMS_DEM_LIB_BIT_EXTRACT','noprompt');
      |         end
      |         set_param([bit_ext_b{:}],'extract_bit','132');
      |     case '_FS(Hold at Key On)'
      |         if ismember(get_param(bit_ext_b,'MaskType'),{'AEMS_DEM_LIB_BIT_EXTRACT'})
      |         else
      |             replace_block(lib_path,'FollowLinks','on','Name','AEMS_DEM_LIB_BIT_EXTRACT','AEMS_Standard_Library/SUB/AEMS_DEM_LIB_BIT_EXTRACT','noprompt');
      |         end
      |         set_param([bit_ext_b{:}],'extract_bit','1');
      |     case '_FS(Reset at Key On)'
      |         if ismember(get_param(bit_ext_b,'MaskType'),{'AEMS_DEM_LIB_BIT_EXTRACT_FS_RESET'})
      |         else
      |             replace_block(lib_path,'FollowLinks','on','Name','AEMS_DEM_LIB_BIT_EXTRACT','AEMS_Standard_Library/SUB/AEMS_DEM_LIB_BIT_EXTRACT_FS_RESET','noprompt');
      |         end
      |         set_param([bit_ext_b{:}],'extract_bit1','1');
      |         set_param([bit_ext_b{:}],'extract_bit2','64');
      |     case '_NBC'
      |         if ismember(get_param(bit_ext_b,'MaskType'),{'AEMS_DEM_LIB_BIT_EXTRACT'})
      |         else
      |             replace_block(lib_path,'FollowLinks','on','Name','AEMS_DEM_LIB_BIT_EXTRACT','AEMS_Standard_Library/SUB/AEMS_DEM_LIB_BIT_EXTRACT','noprompt');
      |         end
      |         set_param([bit_ext_b{:}],'extract_bit','2');
      |     case '_NGBU'
      |         if ismember(get_param(bit_ext_b,'MaskType'),{'AEMS_DEM_LIB_BIT_EXTRACT'})
      |         else
      |             replace_block(lib_path,'FollowLinks','on','Name','AEMS_DEM_LIB_BIT_EXTRACT','AEMS_Standard_Library/SUB/AEMS_DEM_LIB_BIT_EXTRACT','noprompt');
      |         end
      |         set_param([bit_ext_b{:}],'extract_bit','4');
      |     case '_M7NGBU'
      |         if ismember(get_param(bit_ext_b,'MaskType'),{'AEMS_DEM_LIB_BIT_EXTRACT'})
      |         else
      |             replace_block(lib_path,'FollowLinks','on','Name','AEMS_DEM_LIB_BIT_EXTRACT','AEMS_Standard_Library/SUB/AEMS_DEM_LIB_BIT_EXTRACT','noprompt');
      |         end
      |         set_param([bit_ext_b{:}],'extract_bit','4');
      |     case '_NGREM'
      |         if ismember(get_param(bit_ext_b,'MaskType'),{'AEMS_DEM_LIB_BIT_EXTRACT'})
      |         else
      |             replace_block(lib_path,'FollowLinks','on','Name','AEMS_DEM_LIB_BIT_EXTRACT','AEMS_Standard_Library/SUB/AEMS_DEM_LIB_BIT_EXTRACT','noprompt');
      |         end
      |         set_param([bit_ext_b{:}],'extract_bit','8');
      |     case '_NGMEM'
      |         if ismember(get_param(bit_ext_b,'MaskType'),{'AEMS_DEM_LIB_BIT_EXTRACT'})
      |         else
      |             replace_block(lib_path,'FollowLinks','on','Name','AEMS_DEM_LIB_BIT_EXTRACT','AEMS_Standard_Library/SUB/AEMS_DEM_LIB_BIT_EXTRACT','noprompt');
      |         end
      |         set_param([bit_ext_b{:}],'extract_bit','32');
      |     case '_MIL'
      |         if ismember(get_param(bit_ext_b,'MaskType'),{'AEMS_DEM_LIB_BIT_EXTRACT'})
      |         else
      |             replace_block(lib_path,'FollowLinks','on','Name','AEMS_DEM_LIB_BIT_EXTRACT','AEMS_Standard_Library/SUB/AEMS_DEM_LIB_BIT_EXTRACT','noprompt');
      |         end
      |         set_param([bit_ext_b{:}],'extract_bit','128');
      |     case '_FMILON'
      |         if ismember(get_param(bit_ext_b,'MaskType'),{'AEMS_DEM_LIB_BIT_EXTRACT'})
      |         else
      |             replace_block(lib_path,'FollowLinks','on','Name','AEMS_DEM_LIB_BIT_EXTRACT','AEMS_Standard_Library/SUB/AEMS_DEM_LIB_BIT_EXTRACT','noprompt');
      |         end
      |         set_param([bit_ext_b{:}],'extract_bit','128');
      |     case '_FDGNOK'
      |         if ismember(get_param(bit_ext_b,'MaskType'),{'AEMS_DEM_LIB_BIT_EXTRACT_FDGNOK'})
      |         else
      |             replace_block(lib_path,'FollowLinks','on','Name','AEMS_DEM_LIB_BIT_EXTRACT','AEMS_Standard_Library/SUB/AEMS_DEM_LIB_BIT_EXTRACT_FDGNOK','noprompt');
      |         end
      |         set_param([bit_ext_b{:}],'extract_bit1','2');
      |         set_param([bit_ext_b{:}],'extract_bit2','64');
      |     case '_MEM'
      |         if ismember(get_param(bit_ext_b,'MaskType'),{'AEMS_DEM_LIB_BIT_EXTRACT'})
      |         else
      |             replace_block(lib_path,'FollowLinks','on','Name','AEMS_DEM_LIB_BIT_EXTRACT','AEMS_Standard_Library/SUB/AEMS_DEM_LIB_BIT_EXTRACT','noprompt');
      |         end
      |         set_param([bit_ext_b{:}],'extract_bit','32');
      |     case '_FLGMEM'
      |         if ismember(get_param(bit_ext_b,'MaskType'),{'AEMS_DEM_LIB_BIT_EXTRACT'})
      |         else
      |             replace_block(lib_path,'FollowLinks','on','Name','AEMS_DEM_LIB_BIT_EXTRACT','AEMS_Standard_Library/SUB/AEMS_DEM_LIB_BIT_EXTRACT','noprompt');
      |         end
      |         set_param([bit_ext_b{:}],'extract_bit','32');
      | end
      settings: AttributesFormatString=%<MaskType>\nEventId : = %<EventId>\nDEM Library type : = %<LibType>\nFunction Mode : = %<FunctionMode>
      mask TypeOptions LibType: _DGN | _FS(Hold at Key On) | _FS(Reset at Key On) | _NBC | _NGBU | _M7NGBU | _NGREM | _NGMEM | _MIL | _FMILON | _FDGNOK | _MEM | _FLGMEM
      mask TypeOptions FunctionMode: Dysfunctional | From Data Store memory
      mask Display:
      | dgn_mask = ['Event ID: ' char(EventId) '\n Library type: ' char(LibType)];
      | 
      | disp(dgn_mask);
      | plot([5,5,5])
      | plot([6,6,6])
  AEMS_DEM_GET_EVENT_STS_2D : Subsystem  Tag=[LIB]  mask(AEMS_DEM_GET_EVENT_STS_2D){EventId=Dem_EventId_XXX, LibType=_DGN, FunctionMode=Dysfunctional}
      mask prompts: EventId "EventId :"; LibType "DEM Library type :"; FunctionMode "Function Mode"
      mask init:
      | % eval([char(EventId) '_1 = 0;'])
      | % eval([char(EventId) '_2 = 0;'])
      | lib_path = gcb;
      | 
      | Event_Id=get_param(lib_path,'EventId');
      | eventid_b = find_system(lib_path,'LookUnderMasks','all','FollowLinks','on','regexp','on','Name','^EventId_Block');
      | eventid_b1 = find_system(lib_path,'LookUnderMasks','all','FollowLinks','on','Name','EventId_Block1');
      | eval([char(Event_Id) '= 0;']);
      | set_param([eventid_b1{:}],'Value',char(Event_Id));
      | 
      | Splitname=regexp(Event_Id,'_','all');
      | New_EventId=insertBefore(Event_Id,Splitname(end),num2str(2));
      | eval([char(New_EventId) '= 0;']);
      | set_param([eventid_b{2}],'Value',char(New_EventId));
      | 
      | set_param([lib_path,'/AEMS_DEM_GETEVENTSTATUS'],'FunctionMode',FunctionMode);
      | set_param([lib_path,'/AEMS_DEM_GETEVENTSTATUS'],'EventId',char(EventId));
      | set_param([lib_path,'/AEMS_DEM_GETEVENTSTATUS1'],'FunctionMode',FunctionMode);
      | set_param([lib_path,'/AEMS_DEM_GETEVENTSTATUS1'],'EventId',char(New_EventId));
      | 
      | 
      | bit_ext_b1 = find_system(lib_path,'LookUnderMasks','all','FollowLinks','on','Name','DEM_LIB_BIT_EXTRACT1');
      | bit_ext_b2 = find_system(lib_path,'LookUnderMasks','all','FollowLinks','on','Name','DEM_LIB_BIT_EXTRACT2');
      | 
      | switch LibType
      |     case '_DGN'
      |         if ismember(get_param(bit_ext_b1,'MaskType'),{'AEMS_DEM_LIB_BIT_EXTRACT'})
      |         else
      |             replace_block(lib_path,'FollowLinks','on','Name','DEM_LIB_BIT_EXTRACT1','AEMS_Standard_Library/SUB/AEMS_DEM_LIB_BIT_EXTRACT','noprompt');
      |             replace_block(lib_path,'FollowLinks','on','Name','DEM_LIB_BIT_EXTRACT2','AEMS_Standard_Library/SUB/AEMS_DEM_LIB_BIT_EXTRACT','noprompt');
      |         end
      |         set_param([bit_ext_b1{:}],'extract_bit','132');
      |         set_param([bit_ext_b2{:}],'extract_bit','132');
      |     case '_FS(Hold at Key On)'
      |         if ismember(get_param(bit_ext_b1,'MaskType'),{'AEMS_DEM_LIB_BIT_EXTRACT'})
      |         else
      |             replace_block(lib_path,'FollowLinks','on','Name','DEM_LIB_BIT_EXTRACT1','AEMS_Standard_Library/SUB/AEMS_DEM_LIB_BIT_EXTRACT','noprompt');
      |             replace_block(lib_path,'FollowLinks','on','Name','DEM_LIB_BIT_EXTRACT2','AEMS_Standard_Library/SUB/AEMS_DEM_LIB_BIT_EXTRACT','noprompt');
      |         end
      |         set_param([bit_ext_b1{:}],'extract_bit','1');
      |         set_param([bit_ext_b2{:}],'extract_bit','1');
      |     case '_FS(Reset at Key On)'
      |         if ismember(get_param(bit_ext_b1,'MaskType'),{'AEMS_DEM_LIB_BIT_EXTRACT_FS_RESET'})
      |         else
      |             replace_block(lib_path,'FollowLinks','on','Name','DEM_LIB_BIT_EXTRACT1','AEMS_Standard_Library/SUB/AEMS_DEM_LIB_BIT_EXTRACT_FS_RESET','noprompt');
      |             replace_block(lib_path,'FollowLinks','on','Name','DEM_LIB_BIT_EXTRACT2','AEMS_Standard_Library/SUB/AEMS_DEM_LIB_BIT_EXTRACT_FS_RESET','noprompt');
      |         end
      |         set_param([bit_ext_b1{:}],'extract_bit1','1');
      |         set_param([bit_ext_b1{:}],'extract_bit2','64');
      |         set_param([bit_ext_b2{:}],'extract_bit1','1');
      |         set_param([bit_ext_b2{:}],'extract_bit2','64');
      |     case '_NBC'
      |         if ismember(get_param(bit_ext_b1,'MaskType'),{'AEMS_DEM_LIB_BIT_EXTRACT'})
      |         else
      |             replace_block(lib_path,'FollowLinks','on','Name','DEM_LIB_BIT_EXTRACT1','AEMS_Standard_Library/SUB/AEMS_DEM_LIB_BIT_EXTRACT','noprompt');
      |             replace_block(lib_path,'FollowLinks','on','Name','DEM_LIB_BIT_EXTRACT2','AEMS_Standard_Library/SUB/AEMS_DEM_LIB_BIT_EXTRACT','noprompt');
      |         end
      |         set_param([bit_ext_b1{:}],'extract_bit','2');
      |         set_param([bit_ext_b2{:}],'extract_bit','2');
      |     case '_NGBU'
      |         if ismember(get_param(bit_ext_b1,'MaskType'),{'AEMS_DEM_LIB_BIT_EXTRACT'})
      |         else
      |             replace_block(lib_path,'FollowLinks','on','Name','DEM_LIB_BIT_EXTRACT1','AEMS_Standard_Library/SUB/AEMS_DEM_LIB_BIT_EXTRACT','noprompt');
      |             replace_block(lib_path,'FollowLinks','on','Name','DEM_LIB_BIT_EXTRACT2','AEMS_Standard_Library/SUB/AEMS_DEM_LIB_BIT_EXTRACT','noprompt');
      |         end
      |         set_param([bit_ext_b1{:}],'extract_bit','4');
      |         set_param([bit_ext_b2{:}],'extract_bit','4');
      |     case '_M7NGBU'
      |         if ismember(get_param(bit_ext_b1,'MaskType'),{'AEMS_DEM_LIB_BIT_EXTRACT'})
      |         else
      |             replace_block(lib_path,'FollowLinks','on','Name','DEM_LIB_BIT_EXTRACT1','AEMS_Standard_Library/SUB/AEMS_DEM_LIB_BIT_EXTRACT','noprompt');
      |             replace_block(lib_path,'FollowLinks','on','Name','DEM_LIB_BIT_EXTRACT2','AEMS_Standard_Library/SUB/AEMS_DEM_LIB_BIT_EXTRACT','noprompt');
      |         end
      |         set_param([bit_ext_b1{:}],'extract_bit','4');
      |         set_param([bit_ext_b2{:}],'extract_bit','4');
      |     case '_NGREM'
      |         if ismember(get_param(bit_ext_b1,'MaskType'),{'AEMS_DEM_LIB_BIT_EXTRACT'})
      |         else
      |             replace_block(lib_path,'FollowLinks','on','Name','DEM_LIB_BIT_EXTRACT1','AEMS_Standard_Library/SUB/AEMS_DEM_LIB_BIT_EXTRACT','noprompt');
      |             replace_block(lib_path,'FollowLinks','on','Name','DEM_LIB_BIT_EXTRACT2','AEMS_Standard_Library/SUB/AEMS_DEM_LIB_BIT_EXTRACT','noprompt');
      |         end
      |         set_param([bit_ext_b1{:}],'extract_bit','8');
      |         set_param([bit_ext_b2{:}],'extract_bit','8');
      |     case '_NGMEM'
      |         if ismember(get_param(bit_ext_b1,'MaskType'),{'AEMS_DEM_LIB_BIT_EXTRACT'})
      |         else
      |             replace_block(lib_path,'FollowLinks','on','Name','DEM_LIB_BIT_EXTRACT1','AEMS_Standard_Library/SUB/AEMS_DEM_LIB_BIT_EXTRACT','noprompt');
      |             replace_block(lib_path,'FollowLinks','on','Name','DEM_LIB_BIT_EXTRACT2','AEMS_Standard_Library/SUB/AEMS_DEM_LIB_BIT_EXTRACT','noprompt');
      |         end
      |         set_param([bit_ext_b1{:}],'extract_bit','32');
      |         set_param([bit_ext_b2{:}],'extract_bit','32');
      |     case '_MIL'
      |         if ismember(get_param(bit_ext_b1,'MaskType'),{'AEMS_DEM_LIB_BIT_EXTRACT'})
      |         else
      |             replace_block(lib_path,'FollowLinks','on','Name','DEM_LIB_BIT_EXTRACT1','AEMS_Standard_Library/SUB/AEMS_DEM_LIB_BIT_EXTRACT','noprompt');
      |             replace_block(lib_path,'FollowLinks','on','Name','DEM_LIB_BIT_EXTRACT2','AEMS_Standard_Library/SUB/AEMS_DEM_LIB_BIT_EXTRACT','noprompt');
      |         end
      |         set_param([bit_ext_b1{:}],'extract_bit','128');
      |         set_param([bit_ext_b2{:}],'extract_bit','128');
      |     case '_FMILON'
      |         if ismember(get_param(bit_ext_b1,'MaskType'),{'AEMS_DEM_LIB_BIT_EXTRACT'})
      |         else
      |             replace_block(lib_path,'FollowLinks','on','Name','DEM_LIB_BIT_EXTRACT1','AEMS_Standard_Library/SUB/AEMS_DEM_LIB_BIT_EXTRACT','noprompt');
      |             replace_block(lib_path,'FollowLinks','on','Name','DEM_LIB_BIT_EXTRACT2','AEMS_Standard_Library/SUB/AEMS_DEM_LIB_BIT_EXTRACT','noprompt');
      |         end
      |         set_param([bit_ext_b1{:}],'extract_bit','128');
      |         set_param([bit_ext_b2{:}],'extract_bit','128');
      |     case '_FDGNOK'
      |         if ismember(get_param(bit_ext_b1,'MaskType'),{'AEMS_DEM_LIB_BIT_EXTRACT_FDGNOK'})
      |         else
      |             replace_block(lib_path,'FollowLinks','on','Name','DEM_LIB_BIT_EXTRACT1','AEMS_Standard_Library/SUB/AEMS_DEM_LIB_BIT_EXTRACT_FDGNOK','noprompt');
      |             replace_block(lib_path,'FollowLinks','on','Name','DEM_LIB_BIT_EXTRACT2','AEMS_Standard_Library/SUB/AEMS_DEM_LIB_BIT_EXTRACT_FDGNOK','noprompt');
      |         end
      |         set_param([bit_ext_b1{:}],'extract_bit1','2');
      |         set_param([bit_ext_b1{:}],'extract_bit2','64');
      |         set_param([bit_ext_b2{:}],'extract_bit1','2');
      |         set_param([bit_ext_b2{:}],'extract_bit2','64');
      |     case '_MEM'
      |         if ismember(get_param(bit_ext_b1,'MaskType'),{'AEMS_DEM_LIB_BIT_EXTRACT'})
      |         else
      |             replace_block(lib_path,'FollowLinks','on','Name','DEM_LIB_BIT_EXTRACT1','AEMS_Standard_Library/SUB/AEMS_DEM_LIB_BIT_EXTRACT','noprompt');
      |             replace_block(lib_path,'FollowLinks','on','Name','DEM_LIB_BIT_EXTRACT2','AEMS_Standard_Library/SUB/AEMS_DEM_LIB_BIT_EXTRACT','noprompt');
      |         end
      |         set_param([bit_ext_b1{:}],'extract_bit','32');
      |         set_param([bit_ext_b2{:}],'extract_bit','32');
      |     case '_FLGMEM'
      |         if ismember(get_param(bit_ext_b1,'MaskType'),{'AEMS_DEM_LIB_BIT_EXTRACT'})
      |         else
      |             replace_block(lib_path,'FollowLinks','on','Name','DEM_LIB_BIT_EXTRACT1','AEMS_Standard_Library/SUB/AEMS_DEM_LIB_BIT_EXTRACT','noprompt');
      |             replace_block(lib_path,'FollowLinks','on','Name','DEM_LIB_BIT_EXTRACT2','AEMS_Standard_Library/SUB/AEMS_DEM_LIB_BIT_EXTRACT','noprompt');
      |         end
      |         set_param([bit_ext_b1{:}],'extract_bit','32');
      |         set_param([bit_ext_b2{:}],'extract_bit','32');
      | end
      settings: AttributesFormatString=%<MaskType>\nEventId : = %<EventId>\nDEM Library type : = %<LibType>\nFunction Mode : = %<FunctionMode>
      mask TypeOptions LibType: _DGN | _FS(Hold at Key On) | _FS(Reset at Key On) | _NBC | _NGBU | _M7NGBU | _NGREM | _NGMEM | _MIL | _FMILON | _FDGNOK | _MEM | _FLGMEM
      mask TypeOptions FunctionMode: Dysfunctional | From Data Store memory
      mask Display:
      | dgn_mask = ['Event ID: ' char(EventId) '\n Library type: ' char(LibType)];
      | 
      | disp(dgn_mask);
      | plot([5,5,5])
      | plot([6,6,6])
  AEMS_DEM_GET_EVENT_STS_8D : Subsystem  Tag=[LIB]  mask(AEMS_DEM_GET_EVENT_STS_8D){EventId=Dem_EventId_XXX, LibType=_DGN, FunctionMode=Dysfunctional}
      mask prompts: EventId "EventId :"; LibType "DEM Library type :"; FunctionMode "Function Mode"
      mask init:
      | % eval([char(EventId) '_1 = 0;'])
      | % eval([char(EventId) '_2 = 0;'])
      | % eval([char(EventId) '_3 = 0;'])
      | % eval([char(EventId) '_4 = 0;'])
      | % eval([char(EventId) '_5 = 0;'])
      | % eval([char(EventId) '_6 = 0;'])
      | % eval([char(EventId) '_7 = 0;'])
      | % eval([char(EventId) '_8 = 0;'])
      | 
      | lib_path = gcb;
      | Event_Id=get_param(gcb,'EventId');
      | set_param([lib_path,'/AEMS_DEM_GETEVENTSTATUS1'],'EventId',char(Event_Id));
      | set_param([lib_path,'/AEMS_DEM_GETEVENTSTATUS1'],'FunctionMode',FunctionMode);
      | 
      | eventid_b = find_system(gcb,'LookUnderMasks','all','FollowLinks','on','regexp','on','Name','^EventId_Block');
      | eventid_b1 = find_system(gcb,'LookUnderMasks','all','FollowLinks','on','Name','EventId_Block1');
      | eval([char(Event_Id) '= 0;']);
      | set_param(eventid_b1{:},'Value',char(Event_Id));
      | 
      | for len=2:length(eventid_b)
      |     Splitname=regexp(Event_Id,'_','all');
      |     New_EventId=insertBefore(Event_Id,Splitname(end),num2str(len));
      |     eval([char(New_EventId) '= 0;']);
      |     set_param([eventid_b{len}],'Value',char(New_EventId));
      |     set_param([lib_path,['/AEMS_DEM_GETEVENTSTATUS' num2str(len)]],'EventId',char(New_EventId));
      |     set_param([lib_path,['/AEMS_DEM_GETEVENTSTATUS' num2str(len)]],'FunctionMode',FunctionMode);
      | end
      | 
      | % eventid_b1 = find_system(lib_path,'LookUnderMasks','all','FollowLinks','on','Name','EventId_Block1');
      | % eventid_b2 = find_system(lib_path,'LookUnderMasks','all','FollowLinks','on','Name','EventId_Block2');
      | % eventid_b3 = find_system(lib_path,'LookUnderMasks','all','FollowLinks','on','Name','EventId_Block3');
      | % eventid_b4 = find_system(lib_path,'LookUnderMasks','all','FollowLinks','on','Name','EventId_Block4');
      | % eventid_b5 = find_system(lib_path,'LookUnderMasks','all','FollowLinks','on','Name','EventId_Block5');
      | % eventid_b6 = find_system(lib_path,'LookUnderMasks','all','FollowLinks','on','Name','EventId_Block6');
      | % eventid_b7 = find_system(lib_path,'LookUnderMasks','all','FollowLinks','on','Name','EventId_Block7');
      | % eventid_b8 = find_system(lib_path,'LookUnderMasks','all','FollowLinks','on','Name','EventId_Block8');
      | % 
      | % set_param([eventid_b1{:}],'Value',[char(EventId) '_1']);
      | % set_param([eventid_b2{:}],'Value',[char(EventId) '_2']);
      | % set_param([eventid_b3{:}],'Value',[char(EventId) '_3']);
      | % set_param([eventid_b4{:}],'Value',[char(EventId) '_4']);
      | % set_param([eventid_b5{:}],'Value',[char(EventId) '_5']);
      | % set_param([eventid_b6{:}],'Value',[char(EventId) '_6']);
      | % set_param([eventid_b7{:}],'Value',[char(EventId) '_7']);
      | % set_param([eventid_b8{:}],'Value',[char(EventId) '_8']);
      | 
      | bit_ext_b1 = find_system(lib_path,'LookUnderMasks','all','FollowLinks','on','Name','DEM_LIB_BIT_EXTRACT1');
      | bit_ext_b2 = find_system(lib_path,'LookUnderMasks','all','FollowLinks','on','Name','DEM_LIB_BIT_EXTRACT2');
      | bit_ext_b3 = find_system(lib_path,'LookUnderMasks','all','FollowLinks','on','Name','DEM_LIB_BIT_EXTRACT3');
      | bit_ext_b4 = find_system(lib_path,'LookUnderMasks','all','FollowLinks','on','Name','DEM_LIB_BIT_EXTRACT4');
      | bit_ext_b5 = find_system(lib_path,'LookUnderMasks','all','FollowLinks','on','Name','DEM_LIB_BIT_EXTRACT5');
      | bit_ext_b6 = find_system(lib_path,'LookUnderMasks','all','FollowLinks','on','Name','DEM_LIB_BIT_EXTRACT6');
      | bit_ext_b7 = find_system(lib_path,'LookUnderMasks','all','FollowLinks','on','Name','DEM_LIB_BIT_EXTRACT7');
      | bit_ext_b8 = find_system(lib_path,'LookUnderMasks','all','FollowLinks','on','Name','DEM_LIB_BIT_EXTRACT8');
      | 
      | switch LibType
      |     case '_DGN'
      |         if ismember(get_param(bit_ext_b1,'MaskType'),{'AEMS_DEM_LIB_BIT_EXTRACT'})
      |         else
      |             replace_block(lib_path,'FollowLinks','on','Name','DEM_LIB_BIT_EXTRACT1','AEMS_Standard_Library/SUB/AEMS_DEM_LIB_BIT_EXTRACT','noprompt');
      |             replace_block(lib_path,'FollowLinks','on','Name','DEM_LIB_BIT_EXTRACT2','AEMS_Standard_Library/SUB/AEMS_DEM_LIB_BIT_EXTRACT','noprompt');
      |             replace_block(lib_path,'FollowLinks','on','Name','DEM_LIB_BIT_EXTRACT3','AEMS_Standard_Library/SUB/AEMS_DEM_LIB_BIT_EXTRACT','noprompt');
      |             replace_block(lib_path,'FollowLinks','on','Name','DEM_LIB_BIT_EXTRACT4','AEMS_Standard_Library/SUB/AEMS_DEM_LIB_BIT_EXTRACT','noprompt');
      |             replace_block(lib_path,'FollowLinks','on','Name','DEM_LIB_BIT_EXTRACT5','AEMS_Standard_Library/SUB/AEMS_DEM_LIB_BIT_EXTRACT','noprompt');
      |             replace_block(lib_path,'FollowLinks','on','Name','DEM_LIB_BIT_EXTRACT6','AEMS_Standard_Library/SUB/AEMS_DEM_LIB_BIT_EXTRACT','noprompt');
      |             replace_block(lib_path,'FollowLinks','on','Name','DEM_LIB_BIT_EXTRACT7','AEMS_Standard_Library/SUB/AEMS_DEM_LIB_BIT_EXTRACT','noprompt');
      |             replace_block(lib_path,'FollowLinks','on','Name','DEM_LIB_BIT_EXTRACT8','AEMS_Standard_Library/SUB/AEMS_DEM_LIB_BIT_EXTRACT','noprompt');
      |         end
      |         set_param([bit_ext_b1{:}],'extract_bit','132');
      |         set_param([bit_ext_b2{:}],'extract_bit','132');
      |         set_param([bit_ext_b3{:}],'extract_bit','132');
      |         set_param([bit_ext_b4{:}],'extract_bit','132');
      |         set_param([bit_ext_b5{:}],'extract_bit','132');
      |         set_param([bit_ext_b6{:}],'extract_bit','132');
      |         set_param([bit_ext_b7{:}],'extract_bit','132');
      |         set_param([bit_ext_b8{:}],'extract_bit','132');
      |     case '_FS(Hold at Key On)'
      |         if ismember(get_param(bit_ext_b1,'MaskType'),{'AEMS_DEM_LIB_BIT_EXTRACT'})
      |         else
      |             replace_block(lib_path,'FollowLinks','on','Name','DEM_LIB_BIT_EXTRACT1','AEMS_Standard_Library/SUB/AEMS_DEM_LIB_BIT_EXTRACT','noprompt');
      |             replace_block(lib_path,'FollowLinks','on','Name','DEM_LIB_BIT_EXTRACT2','AEMS_Standard_Library/SUB/AEMS_DEM_LIB_BIT_EXTRACT','noprompt');
      |             replace_block(lib_path,'FollowLinks','on','Name','DEM_LIB_BIT_EXTRACT3','AEMS_Standard_Library/SUB/AEMS_DEM_LIB_BIT_EXTRACT','noprompt');
      |             replace_block(lib_path,'FollowLinks','on','Name','DEM_LIB_BIT_EXTRACT4','AEMS_Standard_Library/SUB/AEMS_DEM_LIB_BIT_EXTRACT','noprompt');
      |             replace_block(lib_path,'FollowLinks','on','Name','DEM_LIB_BIT_EXTRACT5','AEMS_Standard_Library/SUB/AEMS_DEM_LIB_BIT_EXTRACT','noprompt');
      |             replace_block(lib_path,'FollowLinks','on','Name','DEM_LIB_BIT_EXTRACT6','AEMS_Standard_Library/SUB/AEMS_DEM_LIB_BIT_EXTRACT','noprompt');
      |             replace_block(lib_path,'FollowLinks','on','Name','DEM_LIB_BIT_EXTRACT7','AEMS_Standard_Library/SUB/AEMS_DEM_LIB_BIT_EXTRACT','noprompt');
      |             replace_block(lib_path,'FollowLinks','on','Name','DEM_LIB_BIT_EXTRACT8','AEMS_Standard_Library/SUB/AEMS_DEM_LIB_BIT_EXTRACT','noprompt');
      |         end
      |         set_param([bit_ext_b1{:}],'extract_bit','1');
      |         set_param([bit_ext_b2{:}],'extract_bit','1');
      |         set_param([bit_ext_b3{:}],'extract_bit','1');
      |         set_param([bit_ext_b4{:}],'extract_bit','1');
      |         set_param([bit_ext_b5{:}],'extract_bit','1');
      |         set_param([bit_ext_b6{:}],'extract_bit','1');
      |         set_param([bit_ext_b7{:}],'extract_bit','1');
      |         set_param([bit_ext_b8{:}],'extract_bit','1');
      |     case '_FS(Reset at Key On)'
      |         if ismember(get_param(bit_ext_b1,'MaskType'),{'AEMS_DEM_LIB_BIT_EXTRACT_FS_RESET'})
      |         else
      |             replace_block(lib_path,'FollowLinks','on','Name','DEM_LIB_BIT_EXTRACT1','AEMS_Standard_Library/SUB/AEMS_DEM_LIB_BIT_EXTRACT_FS_RESET','noprompt');
      |             replace_block(lib_path,'FollowLinks','on','Name','DEM_LIB_BIT_EXTRACT2','AEMS_Standard_Library/SUB/AEMS_DEM_LIB_BIT_EXTRACT_FS_RESET','noprompt');
      |             replace_block(lib_path,'FollowLinks','on','Name','DEM_LIB_BIT_EXTRACT3','AEMS_Standard_Library/SUB/AEMS_DEM_LIB_BIT_EXTRACT_FS_RESET','noprompt');
      |             replace_block(lib_path,'FollowLinks','on','Name','DEM_LIB_BIT_EXTRACT4','AEMS_Standard_Library/SUB/AEMS_DEM_LIB_BIT_EXTRACT_FS_RESET','noprompt');
      |             replace_block(lib_path,'FollowLinks','on','Name','DEM_LIB_BIT_EXTRACT5','AEMS_Standard_Library/SUB/AEMS_DEM_LIB_BIT_EXTRACT_FS_RESET','noprompt');
      |             replace_block(lib_path,'FollowLinks','on','Name','DEM_LIB_BIT_EXTRACT6','AEMS_Standard_Library/SUB/AEMS_DEM_LIB_BIT_EXTRACT_FS_RESET','noprompt');
      |             replace_block(lib_path,'FollowLinks','on','Name','DEM_LIB_BIT_EXTRACT7','AEMS_Standard_Library/SUB/AEMS_DEM_LIB_BIT_EXTRACT_FS_RESET','noprompt');
      |             replace_block(lib_path,'FollowLinks','on','Name','DEM_LIB_BIT_EXTRACT8','AEMS_Standard_Library/SUB/AEMS_DEM_LIB_BIT_EXTRACT_FS_RESET','noprompt');
      |         end
      |         set_param([bit_ext_b1{:}],'extract_bit1','1');
      |         set_param([bit_ext_b1{:}],'extract_bit2','64');
      |         set_param([bit_ext_b2{:}],'extract_bit1','1');
      |         set_param([bit_ext_b2{:}],'extract_bit2','64');
      |         set_param([bit_ext_b3{:}],'extract_bit1','1');
      |         set_param([bit_ext_b3{:}],'extract_bit2','64');
      |         set_param([bit_ext_b4{:}],'extract_bit1','1');
      |         set_param([bit_ext_b4{:}],'extract_bit2','64');
      |         set_param([bit_ext_b5{:}],'extract_bit1','1');
      |         set_param([bit_ext_b5{:}],'extract_bit2','64');
      |         set_param([bit_ext_b6{:}],'extract_bit1','1');
      |         set_param([bit_ext_b6{:}],'extract_bit2','64');
      |         set_param([bit_ext_b7{:}],'extract_bit1','1');
      |         set_param([bit_ext_b7{:}],'extract_bit2','64');
      |         set_param([bit_ext_b8{:}],'extract_bit1','1');
      |         set_param([bit_ext_b8{:}],'extract_bit2','64');
      |     case '_NBC'
      |         if ismember(get_param(bit_ext_b1,'MaskType'),{'AEMS_DEM_LIB_BIT_EXTRACT'})
      |         else
      |             replace_block(lib_path,'FollowLinks','on','Name','DEM_LIB_BIT_EXTRACT1','AEMS_Standard_Library/SUB/AEMS_DEM_LIB_BIT_EXTRACT','noprompt');
      |             replace_block(lib_path,'FollowLinks','on','Name','DEM_LIB_BIT_EXTRACT2','AEMS_Standard_Library/SUB/AEMS_DEM_LIB_BIT_EXTRACT','noprompt');
      |             replace_block(lib_path,'FollowLinks','on','Name','DEM_LIB_BIT_EXTRACT3','AEMS_Standard_Library/SUB/AEMS_DEM_LIB_BIT_EXTRACT','noprompt');
      |             replace_block(lib_path,'FollowLinks','on','Name','DEM_LIB_BIT_EXTRACT4','AEMS_Standard_Library/SUB/AEMS_DEM_LIB_BIT_EXTRACT','noprompt');
      |             replace_block(lib_path,'FollowLinks','on','Name','DEM_LIB_BIT_EXTRACT5','AEMS_Standard_Library/SUB/AEMS_DEM_LIB_BIT_EXTRACT','noprompt');
      |             replace_block(lib_path,'FollowLinks','on','Name','DEM_LIB_BIT_EXTRACT6','AEMS_Standard_Library/SUB/AEMS_DEM_LIB_BIT_EXTRACT','noprompt');
      |             replace_block(lib_path,'FollowLinks','on','Name','DEM_LIB_BIT_EXTRACT7','AEMS_Standard_Library/SUB/AEMS_DEM_LIB_BIT_EXTRACT','noprompt');
      |             replace_block(lib_path,'FollowLinks','on','Name','DEM_LIB_BIT_EXTRACT8','AEMS_Standard_Library/SUB/AEMS_DEM_LIB_BIT_EXTRACT','noprompt');
      |         end
      |         set_param([bit_ext_b1{:}],'extract_bit','2');
      |         set_param([bit_ext_b2{:}],'extract_bit','2');
      |         set_param([bit_ext_b3{:}],'extract_bit','2');
      |         set_param([bit_ext_b4{:}],'extract_bit','2');
      |         set_param([bit_ext_b5{:}],'extract_bit','2');
      |         set_param([bit_ext_b6{:}],'extract_bit','2');
      |         set_param([bit_ext_b7{:}],'extract_bit','2');
      |         set_param([bit_ext_b8{:}],'extract_bit','2');
      |     case '_NGBU'
      |         if ismember(get_param(bit_ext_b1,'MaskType'),{'AEMS_DEM_LIB_BIT_EXTRACT'})
      |         else
      |             replace_block(lib_path,'FollowLinks','on','Name','DEM_LIB_BIT_EXTRACT1','AEMS_Standard_Library/SUB/AEMS_DEM_LIB_BIT_EXTRACT','noprompt');
      |             replace_block(lib_path,'FollowLinks','on','Name','DEM_LIB_BIT_EXTRACT2','AEMS_Standard_Library/SUB/AEMS_DEM_LIB_BIT_EXTRACT','noprompt');
      |             replace_block(lib_path,'FollowLinks','on','Name','DEM_LIB_BIT_EXTRACT3','AEMS_Standard_Library/SUB/AEMS_DEM_LIB_BIT_EXTRACT','noprompt');
      |             replace_block(lib_path,'FollowLinks','on','Name','DEM_LIB_BIT_EXTRACT4','AEMS_Standard_Library/SUB/AEMS_DEM_LIB_BIT_EXTRACT','noprompt');
      |             replace_block(lib_path,'FollowLinks','on','Name','DEM_LIB_BIT_EXTRACT5','AEMS_Standard_Library/SUB/AEMS_DEM_LIB_BIT_EXTRACT','noprompt');
      |             replace_block(lib_path,'FollowLinks','on','Name','DEM_LIB_BIT_EXTRACT6','AEMS_Standard_Library/SUB/AEMS_DEM_LIB_BIT_EXTRACT','noprompt');
      |             replace_block(lib_path,'FollowLinks','on','Name','DEM_LIB_BIT_EXTRACT7','AEMS_Standard_Library/SUB/AEMS_DEM_LIB_BIT_EXTRACT','noprompt');
      |             replace_block(lib_path,'FollowLinks','on','Name','DEM_LIB_BIT_EXTRACT8','AEMS_Standard_Library/SUB/AEMS_DEM_LIB_BIT_EXTRACT','noprompt');
      |         end
      |         set_param([bit_ext_b1{:}],'extract_bit','4');
      |         set_param([bit_ext_b2{:}],'extract_bit','4');
      |         set_param([bit_ext_b3{:}],'extract_bit','4');
      |         set_param([bit_ext_b4{:}],'extract_bit','4');
      |         set_param([bit_ext_b5{:}],'extract_bit','4');
      |         set_param([bit_ext_b6{:}],'extract_bit','4');
      |         set_param([bit_ext_b7{:}],'extract_bit','4');
      |         set_param([bit_ext_b8{:}],'extract_bit','4');
      |     case '_M7NGBU'
      |         if ismember(get_param(bit_ext_b1,'MaskType'),{'AEMS_DEM_LIB_BIT_EXTRACT'})
      |         else
      |             replace_block(lib_path,'FollowLinks','on','Name','DEM_LIB_BIT_EXTRACT1','AEMS_Standard_Library/SUB/AEMS_DEM_LIB_BIT_EXTRACT','noprompt');
      |             replace_block(lib_path,'FollowLinks','on','Name','DEM_LIB_BIT_EXTRACT2','AEMS_Standard_Library/SUB/AEMS_DEM_LIB_BIT_EXTRACT','noprompt');
      |             replace_block(lib_path,'FollowLinks','on','Name','DEM_LIB_BIT_EXTRACT3','AEMS_Standard_Library/SUB/AEMS_DEM_LIB_BIT_EXTRACT','noprompt');
      |             replace_block(lib_path,'FollowLinks','on','Name','DEM_LIB_BIT_EXTRACT4','AEMS_Standard_Library/SUB/AEMS_DEM_LIB_BIT_EXTRACT','noprompt');
      |             replace_block(lib_path,'FollowLinks','on','Name','DEM_LIB_BIT_EXTRACT5','AEMS_Standard_Library/SUB/AEMS_DEM_LIB_BIT_EXTRACT','noprompt');
      |             replace_block(lib_path,'FollowLinks','on','Name','DEM_LIB_BIT_EXTRACT6','AEMS_Standard_Library/SUB/AEMS_DEM_LIB_BIT_EXTRACT','noprompt');
      |             replace_block(lib_path,'FollowLinks','on','Name','DEM_LIB_BIT_EXTRACT7','AEMS_Standard_Library/SUB/AEMS_DEM_LIB_BIT_EXTRACT','noprompt');
      |             replace_block(lib_path,'FollowLinks','on','Name','DEM_LIB_BIT_EXTRACT8','AEMS_Standard_Library/SUB/AEMS_DEM_LIB_BIT_EXTRACT','noprompt');
      |         end
      |         set_param([bit_ext_b1{:}],'extract_bit','4');
      |         set_param([bit_ext_b2{:}],'extract_bit','4');
      |         set_param([bit_ext_b3{:}],'extract_bit','4');
      |         set_param([bit_ext_b4{:}],'extract_bit','4');
      |         set_param([bit_ext_b5{:}],'extract_bit','4');
      |         set_param([bit_ext_b6{:}],'extract_bit','4');
      |         set_param([bit_ext_b7{:}],'extract_bit','4');
      |         set_param([bit_ext_b8{:}],'extract_bit','4');
      |     case '_NGREM'
      |         if ismember(get_param(bit_ext_b1,'MaskType'),{'AEMS_DEM_LIB_BIT_EXTRACT'})
      |         else
      |             replace_block(lib_path,'FollowLinks','on','Name','DEM_LIB_BIT_EXTRACT1','AEMS_Standard_Library/SUB/AEMS_DEM_LIB_BIT_EXTRACT','noprompt');
      |             replace_block(lib_path,'FollowLinks','on','Name','DEM_LIB_BIT_EXTRACT2','AEMS_Standard_Library/SUB/AEMS_DEM_LIB_BIT_EXTRACT','noprompt');
      |             replace_block(lib_path,'FollowLinks','on','Name','DEM_LIB_BIT_EXTRACT3','AEMS_Standard_Library/SUB/AEMS_DEM_LIB_BIT_EXTRACT','noprompt');
      |             replace_block(lib_path,'FollowLinks','on','Name','DEM_LIB_BIT_EXTRACT4','AEMS_Standard_Library/SUB/AEMS_DEM_LIB_BIT_EXTRACT','noprompt');
      |             replace_block(lib_path,'FollowLinks','on','Name','DEM_LIB_BIT_EXTRACT5','AEMS_Standard_Library/SUB/AEMS_DEM_LIB_BIT_EXTRACT','noprompt');
      |             replace_block(lib_path,'FollowLinks','on','Name','DEM_LIB_BIT_EXTRACT6','AEMS_Standard_Library/SUB/AEMS_DEM_LIB_BIT_EXTRACT','noprompt');
      |             replace_block(lib_path,'FollowLinks','on','Name','DEM_LIB_BIT_EXTRACT7','AEMS_Standard_Library/SUB/AEMS_DEM_LIB_BIT_EXTRACT','noprompt');
      |             replace_block(lib_path,'FollowLinks','on','Name','DEM_LIB_BIT_EXTRACT8','AEMS_Standard_Library/SUB/AEMS_DEM_LIB_BIT_EXTRACT','noprompt');
      |         end
      |         set_param([bit_ext_b1{:}],'extract_bit','8');
      |         set_param([bit_ext_b2{:}],'extract_bit','8');
      |         set_param([bit_ext_b3{:}],'extract_bit','8');
      |         set_param([bit_ext_b4{:}],'extract_bit','8');
      |         set_param([bit_ext_b5{:}],'extract_bit','8');
      |         set_param([bit_ext_b6{:}],'extract_bit','8');
      |         set_param([bit_ext_b7{:}],'extract_bit','8');
      |         set_param([bit_ext_b8{:}],'extract_bit','8');
      |     case '_NGMEM'
      |         if ismember(get_param(bit_ext_b1,'MaskType'),{'AEMS_DEM_LIB_BIT_EXTRACT'})
      |         else
      |             replace_block(lib_path,'FollowLinks','on','Name','DEM_LIB_BIT_EXTRACT1','AEMS_Standard_Library/SUB/AEMS_DEM_LIB_BIT_EXTRACT','noprompt');
      |             replace_block(lib_path,'FollowLinks','on','Name','DEM_LIB_BIT_EXTRACT2','AEMS_Standard_Library/SUB/AEMS_DEM_LIB_BIT_EXTRACT','noprompt');
      |             replace_block(lib_path,'FollowLinks','on','Name','DEM_LIB_BIT_EXTRACT3','AEMS_Standard_Library/SUB/AEMS_DEM_LIB_BIT_EXTRACT','noprompt');
      |             replace_block(lib_path,'FollowLinks','on','Name','DEM_LIB_BIT_EXTRACT4','AEMS_Standard_Library/SUB/AEMS_DEM_LIB_BIT_EXTRACT','noprompt');
      |             replace_block(lib_path,'FollowLinks','on','Name','DEM_LIB_BIT_EXTRACT5','AEMS_Standard_Library/SUB/AEMS_DEM_LIB_BIT_EXTRACT','noprompt');
      |             replace_block(lib_path,'FollowLinks','on','Name','DEM_LIB_BIT_EXTRACT6','AEMS_Standard_Library/SUB/AEMS_DEM_LIB_BIT_EXTRACT','noprompt');
      |             replace_block(lib_path,'FollowLinks','on','Name','DEM_LIB_BIT_EXTRACT7','AEMS_Standard_Library/SUB/AEMS_DEM_LIB_BIT_EXTRACT','noprompt');
      |             replace_block(lib_path,'FollowLinks','on','Name','DEM_LIB_BIT_EXTRACT8','AEMS_Standard_Library/SUB/AEMS_DEM_LIB_BIT_EXTRACT','noprompt');
      |         end
      |         set_param([bit_ext_b1{:}],'extract_bit','32');
      |         set_param([bit_ext_b2{:}],'extract_bit','32');
      |         set_param([bit_ext_b3{:}],'extract_bit','32');
      |         set_param([bit_ext_b4{:}],'extract_bit','32');
      |         set_param([bit_ext_b5{:}],'extract_bit','32');
      |         set_param([bit_ext_b6{:}],'extract_bit','32');
      |         set_param([bit_ext_b7{:}],'extract_bit','32');
      |         set_param([bit_ext_b8{:}],'extract_bit','32');
      |     case '_MIL'
      |         if ismember(get_param(bit_ext_b1,'MaskType'),{'AEMS_DEM_LIB_BIT_EXTRACT'})
      |         else
      |             replace_block(lib_path,'FollowLinks','on','Name','DEM_LIB_BIT_EXTRACT1','AEMS_Standard_Library/SUB/AEMS_DEM_LIB_BIT_EXTRACT','noprompt');
      |             replace_block(lib_path,'FollowLinks','on','Name','DEM_LIB_BIT_EXTRACT2','AEMS_Standard_Library/SUB/AEMS_DEM_LIB_BIT_EXTRACT','noprompt');
      |             replace_block(lib_path,'FollowLinks','on','Name','DEM_LIB_BIT_EXTRACT3','AEMS_Standard_Library/SUB/AEMS_DEM_LIB_BIT_EXTRACT','noprompt');
      |             replace_block(lib_path,'FollowLinks','on','Name','DEM_LIB_BIT_EXTRACT4','AEMS_Standard_Library/SUB/AEMS_DEM_LIB_BIT_EXTRACT','noprompt');
      |             replace_block(lib_path,'FollowLinks','on','Name','DEM_LIB_BIT_EXTRACT5','AEMS_Standard_Library/SUB/AEMS_DEM_LIB_BIT_EXTRACT','noprompt');
      |             replace_block(lib_path,'FollowLinks','on','Name','DEM_LIB_BIT_EXTRACT6','AEMS_Standard_Library/SUB/AEMS_DEM_LIB_BIT_EXTRACT','noprompt');
      |             replace_block(lib_path,'FollowLinks','on','Name','DEM_LIB_BIT_EXTRACT7','AEMS_Standard_Library/SUB/AEMS_DEM_LIB_BIT_EXTRACT','noprompt');
      |             replace_block(lib_path,'FollowLinks','on','Name','DEM_LIB_BIT_EXTRACT8','AEMS_Standard_Library/SUB/AEMS_DEM_LIB_BIT_EXTRACT','noprompt');
      |         end
      |         set_param([bit_ext_b1{:}],'extract_bit','128');
      |         set_param([bit_ext_b2{:}],'extract_bit','128');
      |         set_param([bit_ext_b3{:}],'extract_bit','128');
      |         set_param([bit_ext_b4{:}],'extract_bit','128');
      |         set_param([bit_ext_b5{:}],'extract_bit','128');
      |         set_param([bit_ext_b6{:}],'extract_bit','128');
      |         set_param([bit_ext_b7{:}],'extract_bit','128');
      |         set_param([bit_ext_b8{:}],'extract_bit','128');
      |     case '_FMILON'
      |         if ismember(get_param(bit_ext_b1,'MaskType'),{'AEMS_DEM_LIB_BIT_EXTRACT'})
      |         else
      |             replace_block(lib_path,'FollowLinks','on','Name','DEM_LIB_BIT_EXTRACT1','AEMS_Standard_Library/SUB/AEMS_DEM_LIB_BIT_EXTRACT','noprompt');
      |             replace_block(lib_path,'FollowLinks','on','Name','DEM_LIB_BIT_EXTRACT2','AEMS_Standard_Library/SUB/AEMS_DEM_LIB_BIT_EXTRACT','noprompt');
      |             replace_block(lib_path,'FollowLinks','on','Name','DEM_LIB_BIT_EXTRACT3','AEMS_Standard_Library/SUB/AEMS_DEM_LIB_BIT_EXTRACT','noprompt');
      |             replace_block(lib_path,'FollowLinks','on','Name','DEM_LIB_BIT_EXTRACT4','AEMS_Standard_Library/SUB/AEMS_DEM_LIB_BIT_EXTRACT','noprompt');
      |             replace_block(lib_path,'FollowLinks','on','Name','DEM_LIB_BIT_EXTRACT5','AEMS_Standard_Library/SUB/AEMS_DEM_LIB_BIT_EXTRACT','noprompt');
      |             replace_block(lib_path,'FollowLinks','on','Name','DEM_LIB_BIT_EXTRACT6','AEMS_Standard_Library/SUB/AEMS_DEM_LIB_BIT_EXTRACT','noprompt');
      |             replace_block(lib_path,'FollowLinks','on','Name','DEM_LIB_BIT_EXTRACT7','AEMS_Standard_Library/SUB/AEMS_DEM_LIB_BIT_EXTRACT','noprompt');
      |             replace_block(lib_path,'FollowLinks','on','Name','DEM_LIB_BIT_EXTRACT8','AEMS_Standard_Library/SUB/AEMS_DEM_LIB_BIT_EXTRACT','noprompt');
      |         end
      |         set_param([bit_ext_b1{:}],'extract_bit','128');
      |         set_param([bit_ext_b2{:}],'extract_bit','128');
      |         set_param([bit_ext_b3{:}],'extract_bit','128');
      |         set_param([bit_ext_b4{:}],'extract_bit','128');
      |         set_param([bit_ext_b5{:}],'extract_bit','128');
      |         set_param([bit_ext_b6{:}],'extract_bit','128');
      |         set_param([bit_ext_b7{:}],'extract_bit','128');
      |         set_param([bit_ext_b8{:}],'extract_bit','128');
      |     case '_FDGNOK'
      |         if ismember(get_param(bit_ext_b1,'MaskType'),{'AEMS_DEM_LIB_BIT_EXTRACT_FDGNOK'})
      |         else
      |             replace_block(lib_path,'FollowLinks','on','Name','DEM_LIB_BIT_EXTRACT1','AEMS_Standard_Library/SUB/AEMS_DEM_LIB_BIT_EXTRACT_FDGNOK','noprompt');
      |             replace_block(lib_path,'FollowLinks','on','Name','DEM_LIB_BIT_EXTRACT2','AEMS_Standard_Library/SUB/AEMS_DEM_LIB_BIT_EXTRACT_FDGNOK','noprompt');
      |             replace_block(lib_path,'FollowLinks','on','Name','DEM_LIB_BIT_EXTRACT3','AEMS_Standard_Library/SUB/AEMS_DEM_LIB_BIT_EXTRACT_FDGNOK','noprompt');
      |             replace_block(lib_path,'FollowLinks','on','Name','DEM_LIB_BIT_EXTRACT4','AEMS_Standard_Library/SUB/AEMS_DEM_LIB_BIT_EXTRACT_FDGNOK','noprompt');
      |             replace_block(lib_path,'FollowLinks','on','Name','DEM_LIB_BIT_EXTRACT5','AEMS_Standard_Library/SUB/AEMS_DEM_LIB_BIT_EXTRACT_FDGNOK','noprompt');
      |             replace_block(lib_path,'FollowLinks','on','Name','DEM_LIB_BIT_EXTRACT6','AEMS_Standard_Library/SUB/AEMS_DEM_LIB_BIT_EXTRACT_FDGNOK','noprompt');
      |             replace_block(lib_path,'FollowLinks','on','Name','DEM_LIB_BIT_EXTRACT7','AEMS_Standard_Library/SUB/AEMS_DEM_LIB_BIT_EXTRACT_FDGNOK','noprompt');
      |             replace_block(lib_path,'FollowLinks','on','Name','DEM_LIB_BIT_EXTRACT8','AEMS_Standard_Library/SUB/AEMS_DEM_LIB_BIT_EXTRACT_FDGNOK','noprompt');
      |         end
      |         set_param([bit_ext_b1{:}],'extract_bit1','2');
      |         set_param([bit_ext_b1{:}],'extract_bit2','64');
      |         set_param([bit_ext_b2{:}],'extract_bit1','2');
      |         set_param([bit_ext_b2{:}],'extract_bit2','64');
      |         set_param([bit_ext_b3{:}],'extract_bit1','2');
      |         set_param([bit_ext_b3{:}],'extract_bit2','64');
      |         set_param([bit_ext_b4{:}],'extract_bit1','2');
      |         set_param([bit_ext_b4{:}],'extract_bit2','64');
      |         set_param([bit_ext_b5{:}],'extract_bit1','2');
      |         set_param([bit_ext_b5{:}],'extract_bit2','64');
      |         set_param([bit_ext_b6{:}],'extract_bit1','2');
      |         set_param([bit_ext_b6{:}],'extract_bit2','64');
      |         set_param([bit_ext_b7{:}],'extract_bit1','2');
      |         set_param([bit_ext_b7{:}],'extract_bit2','64');
      |         set_param([bit_ext_b8{:}],'extract_bit1','2');
      |         set_param([bit_ext_b8{:}],'extract_bit2','64');
      |     case '_MEM'
      |         if ismember(get_param(bit_ext_b1,'MaskType'),{'AEMS_DEM_LIB_BIT_EXTRACT'})
      |         else
      |             replace_block(lib_path,'FollowLinks','on','Name','DEM_LIB_BIT_EXTRACT1','AEMS_Standard_Library/SUB/AEMS_DEM_LIB_BIT_EXTRACT','noprompt');
      |             replace_block(lib_path,'FollowLinks','on','Name','DEM_LIB_BIT_EXTRACT2','AEMS_Standard_Library/SUB/AEMS_DEM_LIB_BIT_EXTRACT','noprompt');
      |             replace_block(lib_path,'FollowLinks','on','Name','DEM_LIB_BIT_EXTRACT3','AEMS_Standard_Library/SUB/AEMS_DEM_LIB_BIT_EXTRACT','noprompt');
      |             replace_block(lib_path,'FollowLinks','on','Name','DEM_LIB_BIT_EXTRACT4','AEMS_Standard_Library/SUB/AEMS_DEM_LIB_BIT_EXTRACT','noprompt');
      |             replace_block(lib_path,'FollowLinks','on','Name','DEM_LIB_BIT_EXTRACT5','AEMS_Standard_Library/SUB/AEMS_DEM_LIB_BIT_EXTRACT','noprompt');
      |             replace_block(lib_path,'FollowLinks','on','Name','DEM_LIB_BIT_EXTRACT6','AEMS_Standard_Library/SUB/AEMS_DEM_LIB_BIT_EXTRACT','noprompt');
      |             replace_block(lib_path,'FollowLinks','on','Name','DEM_LIB_BIT_EXTRACT7','AEMS_Standard_Library/SUB/AEMS_DEM_LIB_BIT_EXTRACT','noprompt');
      |             replace_block(lib_path,'FollowLinks','on','Name','DEM_LIB_BIT_EXTRACT8','AEMS_Standard_Library/SUB/AEMS_DEM_LIB_BIT_EXTRACT','noprompt');
      |         end
      |         set_param([bit_ext_b1{:}],'extract_bit','32');
      |         set_param([bit_ext_b2{:}],'extract_bit','32');
      |         set_param([bit_ext_b3{:}],'extract_bit','32');
      |         set_param([bit_ext_b4{:}],'extract_bit','32');
      |         set_param([bit_ext_b5{:}],'extract_bit','32');
      |         set_param([bit_ext_b6{:}],'extract_bit','32');
      |         set_param([bit_ext_b7{:}],'extract_bit','32');
      |         set_param([bit_ext_b8{:}],'extract_bit','32');
      |     case '_FLGMEM'
      |         if ismember(get_param(bit_ext_b1,'MaskType'),{'AEMS_DEM_LIB_BIT_EXTRACT'})
      |         else
      |             replace_block(lib_path,'FollowLinks','on','Name','DEM_LIB_BIT_EXTRACT1','AEMS_Standard_Library/SUB/AEMS_DEM_LIB_BIT_EXTRACT','noprompt');
      |             replace_block(lib_path,'FollowLinks','on','Name','DEM_LIB_BIT_EXTRACT2','AEMS_Standard_Library/SUB/AEMS_DEM_LIB_BIT_EXTRACT','noprompt');
      |             replace_block(lib_path,'FollowLinks','on','Name','DEM_LIB_BIT_EXTRACT3','AEMS_Standard_Library/SUB/AEMS_DEM_LIB_BIT_EXTRACT','noprompt');
      |             replace_block(lib_path,'FollowLinks','on','Name','DEM_LIB_BIT_EXTRACT4','AEMS_Standard_Library/SUB/AEMS_DEM_LIB_BIT_EXTRACT','noprompt');
      |             replace_block(lib_path,'FollowLinks','on','Name','DEM_LIB_BIT_EXTRACT5','AEMS_Standard_Library/SUB/AEMS_DEM_LIB_BIT_EXTRACT','noprompt');
      |             replace_block(lib_path,'FollowLinks','on','Name','DEM_LIB_BIT_EXTRACT6','AEMS_Standard_Library/SUB/AEMS_DEM_LIB_BIT_EXTRACT','noprompt');
      |             replace_block(lib_path,'FollowLinks','on','Name','DEM_LIB_BIT_EXTRACT7','AEMS_Standard_Library/SUB/AEMS_DEM_LIB_BIT_EXTRACT','noprompt');
      |             replace_block(lib_path,'FollowLinks','on','Name','DEM_LIB_BIT_EXTRACT8','AEMS_Standard_Library/SUB/AEMS_DEM_LIB_BIT_EXTRACT','noprompt');
      |         end
      |         set_param([bit_ext_b1{:}],'extract_bit','32');
      |         set_param([bit_ext_b2{:}],'extract_bit','32');
      |         set_param([bit_ext_b3{:}],'extract_bit','32');
      |         set_param([bit_ext_b4{:}],'extract_bit','32');
      |         set_param([bit_ext_b5{:}],'extract_bit','32');
      |         set_param([bit_ext_b6{:}],'extract_bit','32');
      |         set_param([bit_ext_b7{:}],'extract_bit','32');
      |         set_param([bit_ext_b8{:}],'extract_bit','32');
      | end
      settings: AttributesFormatString=%<MaskType>\nEventId : = %<EventId>\nDEM Library type : = %<LibType>\nFunction Mode : = %<FunctionMode>
      mask TypeOptions LibType: _DGN | _FS(Hold at Key On) | _FS(Reset at Key On) | _NBC | _NGBU | _M7NGBU | _NGREM | _NGMEM | _MIL | _FMILON | _FDGNOK | _MEM | _FLGMEM
      mask TypeOptions FunctionMode: Dysfunctional | From Data Store memory
      mask Display:
      | dgn_mask = ['Event ID: ' char(EventId) '\n Library type: ' char(LibType)];
      | 
      | disp(dgn_mask);
      | plot([5,5,5])
      | plot([6,6,6])
  AEMS_DEM_GET_EVENT_STS_9D : Subsystem  Tag=[LIB]  mask(AEMS_DEM_GET_EVENT_STS_9D){EventId=Dem_EventId_XXX, LibType=_DGN, FunctionMode=Dysfunctional}
      mask prompts: EventId "EventId :"; LibType "DEM Library type :"; FunctionMode "Function Mode"
      mask init:
      | % eval([char(EventId) '_1 = 0;'])
      | % eval([char(EventId) '_2 = 0;'])
      | % eval([char(EventId) '_3 = 0;'])
      | % eval([char(EventId) '_4 = 0;'])
      | % eval([char(EventId) '_5 = 0;'])
      | % eval([char(EventId) '_6 = 0;'])
      | % eval([char(EventId) '_7 = 0;'])
      | % eval([char(EventId) '_8 = 0;'])
      | % eval([char(EventId) '_0 = 0;'])
      | 
      | lib_path = gcb;
      | Event_Id=get_param(gcb,'EventId');
      | 
      | set_param([lib_path,'/AEMS_DEM_GETEVENTSTATUS1'],'EventId',char(Event_Id));
      | set_param([lib_path,'/AEMS_DEM_GETEVENTSTATUS1'],'FunctionMode',FunctionMode);
      | 
      | eventid_b = find_system(gcb,'LookUnderMasks','all','FollowLinks','on','regexp','on','Name','^EventId_Block');
      | eventid_b1 = find_system(gcb,'LookUnderMasks','all','FollowLinks','on','Name','EventId_Block0');
      | eval([char(Event_Id) '= 0;']);
      | set_param(eventid_b1{:},'Value',char(Event_Id));
      | 
      | for len=2:length(eventid_b)
      |     Splitname=regexp(Event_Id,'_','all');
      |     New_EventId=insertBefore(Event_Id,Splitname(end),num2str(len));
      |     eval([char(New_EventId) '= 0;']);
      |     set_param([eventid_b{len}],'Value',char(New_EventId));
      |     set_param([lib_path,['/AEMS_DEM_GETEVENTSTATUS' num2str(len)]],'EventId',char(New_EventId));
      |     set_param([lib_path,['/AEMS_DEM_GETEVENTSTATUS' num2str(len)]],'FunctionMode',FunctionMode);
      | end
      | % eventid_b1 = find_system(lib_path,'LookUnderMasks','all','FollowLinks','on','Name','EventId_Block1');
      | % eventid_b2 = find_system(lib_path,'LookUnderMasks','all','FollowLinks','on','Name','EventId_Block2');
      | % eventid_b3 = find_system(lib_path,'LookUnderMasks','all','FollowLinks','on','Name','EventId_Block3');
      | % eventid_b4 = find_system(lib_path,'LookUnderMasks','all','FollowLinks','on','Name','EventId_Block4');
      | % eventid_b5 = find_system(lib_path,'LookUnderMasks','all','FollowLinks','on','Name','EventId_Block5');
      | % eventid_b6 = find_system(lib_path,'LookUnderMasks','all','FollowLinks','on','Name','EventId_Block6');
      | % eventid_b7 = find_system(lib_path,'LookUnderMasks','all','FollowLinks','on','Name','EventId_Block7');
      | % eventid_b8 = find_system(lib_path,'LookUnderMasks','all','FollowLinks','on','Name','EventId_Block8');
      | % eventid_b0 = find_system(lib_path,'LookUnderMasks','all','FollowLinks','on','Name','EventId_Block0');
      | % 
      | % set_param([eventid_b1{:}],'Value',[char(EventId) '_1']);
      | % set_param([eventid_b2{:}],'Value',[char(EventId) '_2']);
      | % set_param([eventid_b3{:}],'Value',[char(EventId) '_3']);
      | % set_param([eventid_b4{:}],'Value',[char(EventId) '_4']);
      | % set_param([eventid_b5{:}],'Value',[char(EventId) '_5']);
      | % set_param([eventid_b6{:}],'Value',[char(EventId) '_6']);
      | % set_param([eventid_b7{:}],'Value',[char(EventId) '_7']);
      | % set_param([eventid_b8{:}],'Value',[char(EventId) '_8']);
      | % set_param([eventid_b0{:}],'Value',[char(EventId) '_0']);
      | 
      | bit_ext_b1 = find_system(lib_path,'LookUnderMasks','all','FollowLinks','on','Name','DEM_LIB_BIT_EXTRACT1');
      | bit_ext_b2 = find_system(lib_path,'LookUnderMasks','all','FollowLinks','on','Name','DEM_LIB_BIT_EXTRACT2');
      | bit_ext_b3 = find_system(lib_path,'LookUnderMasks','all','FollowLinks','on','Name','DEM_LIB_BIT_EXTRACT3');
      | bit_ext_b4 = find_system(lib_path,'LookUnderMasks','all','FollowLinks','on','Name','DEM_LIB_BIT_EXTRACT4');
      | bit_ext_b5 = find_system(lib_path,'LookUnderMasks','all','FollowLinks','on','Name','DEM_LIB_BIT_EXTRACT5');
      | bit_ext_b6 = find_system(lib_path,'LookUnderMasks','all','FollowLinks','on','Name','DEM_LIB_BIT_EXTRACT6');
